simulink model "model"  (R2016a)
(part 4 of 5)

  bus264 : powerlib/Measurements/Load Flow Bus  LConnTagsString=a  Phases=single  Connectors=on one side  ID=bus264  Vbase=400000  Vref=1  Vangle=0  VLF=1  VLFb=1  VLFc=1  angleLF=0  angleLFb=0  angleLFc=0
      settings: AttributesFormatString=|
      | %<ID>
      | %<Vbase>V
      | %<VLF>pu
      | %<angleLF>deg.
      | %<Name>
  bus265 : powerlib/Measurements/Load Flow Bus  LConnTagsString=a  Phases=single  Connectors=on one side  ID=bus265  Vbase=400000  Vref=1  Vangle=0  VLF=1  VLFb=1  VLFc=1  angleLF=0  angleLFb=0  angleLFc=0
      settings: AttributesFormatString=|
      | %<ID>
      | %<Vbase>V
      | %<VLF>pu
      | %<angleLF>deg.
      | %<Name>
  bus266 : powerlib/Measurements/Load Flow Bus  LConnTagsString=a  Phases=single  Connectors=on one side  ID=bus266  Vbase=400000  Vref=1  Vangle=0  VLF=1  VLFb=1  VLFc=1  angleLF=0  angleLFb=0  angleLFc=0
      settings: AttributesFormatString=|
      | %<ID>
      | %<Vbase>V
      | %<VLF>pu
      | %<angleLF>deg.
      | %<Name>
  bus267 : powerlib/Measurements/Load Flow Bus  LConnTagsString=a  Phases=single  Connectors=on one side  ID=bus267  Vbase=400000  Vref=1  Vangle=0  VLF=1  VLFb=1  VLFc=1  angleLF=0  angleLFb=0  angleLFc=0
      settings: AttributesFormatString=|
      | %<ID>
      | %<Vbase>V
      | %<VLF>pu
      | %<angleLF>deg.
      | %<Name>
  bus268 : powerlib/Measurements/Load Flow Bus  LConnTagsString=a  Phases=single  Connectors=on one side  ID=bus268  Vbase=400000  Vref=1  Vangle=0  VLF=1  VLFb=1  VLFc=1  angleLF=0  angleLFb=0  angleLFc=0
      settings: AttributesFormatString=|
      | %<ID>
      | %<Vbase>V
      | %<VLF>pu
      | %<angleLF>deg.
      | %<Name>
  bus269 : powerlib/Measurements/Load Flow Bus  LConnTagsString=a  Phases=single  Connectors=on one side  ID=bus269  Vbase=400000  Vref=1  Vangle=0  VLF=1  VLFb=1  VLFc=1  angleLF=0  angleLFb=0  angleLFc=0
      settings: AttributesFormatString=|
      | %<ID>
      | %<Vbase>V
      | %<VLF>pu
      | %<angleLF>deg.
      | %<Name>
  bus27 : powerlib/Measurements/Load Flow Bus  LConnTagsString=a  Phases=single  Connectors=on one side  ID=bus27  Vbase=400000  Vref=1  Vangle=0  VLF=1  VLFb=1  VLFc=1  angleLF=0  angleLFb=0  angleLFc=0
      settings: AttributesFormatString=|
      | %<ID>
      | %<Vbase>V
      | %<VLF>pu
      | %<angleLF>deg.
      | %<Name>
  bus270 : powerlib/Measurements/Load Flow Bus  LConnTagsString=a  Phases=single  Connectors=on one side  ID=bus270  Vbase=400000  Vref=1  Vangle=0  VLF=1  VLFb=1  VLFc=1  angleLF=0  angleLFb=0  angleLFc=0
      settings: AttributesFormatString=|
      | %<ID>
      | %<Vbase>V
      | %<VLF>pu
      | %<angleLF>deg.
      | %<Name>
  bus271 : powerlib/Measurements/Load Flow Bus  LConnTagsString=a  Phases=single  Connectors=on one side  ID=bus271  Vbase=400000  Vref=1  Vangle=0  VLF=1  VLFb=1  VLFc=1  angleLF=0  angleLFb=0  angleLFc=0
      settings: AttributesFormatString=|
      | %<ID>
      | %<Vbase>V
      | %<VLF>pu
      | %<angleLF>deg.
      | %<Name>
  bus272 : powerlib/Measurements/Load Flow Bus  LConnTagsString=a  Phases=single  Connectors=on one side  ID=bus272  Vbase=400000  Vref=1  Vangle=0  VLF=1  VLFb=1  VLFc=1  angleLF=0  angleLFb=0  angleLFc=0
      settings: AttributesFormatString=|
      | %<ID>
      | %<Vbase>V
      | %<VLF>pu
      | %<angleLF>deg.
      | %<Name>
  bus273 : powerlib/Measurements/Load Flow Bus  LConnTagsString=a  Phases=single  Connectors=on one side  ID=bus273  Vbase=400000  Vref=1  Vangle=0  VLF=1  VLFb=1  VLFc=1  angleLF=0  angleLFb=0  angleLFc=0
      settings: AttributesFormatString=|
      | %<ID>
      | %<Vbase>V
      | %<VLF>pu
      | %<angleLF>deg.
      | %<Name>
  bus274 : powerlib/Measurements/Load Flow Bus  LConnTagsString=a  Phases=single  Connectors=on one side  ID=bus274  Vbase=400000  Vref=1  Vangle=0  VLF=1  VLFb=1  VLFc=1  angleLF=0  angleLFb=0  angleLFc=0
      settings: AttributesFormatString=|
      | %<ID>
      | %<Vbase>V
      | %<VLF>pu
      | %<angleLF>deg.
      | %<Name>
  bus275 : powerlib/Measurements/Load Flow Bus  LConnTagsString=a  Phases=single  Connectors=on one side  ID=bus275  Vbase=400000  Vref=1  Vangle=0  VLF=1  VLFb=1  VLFc=1  angleLF=0  angleLFb=0  angleLFc=0
      settings: AttributesFormatString=|
      | %<ID>
      | %<Vbase>V
      | %<VLF>pu
      | %<angleLF>deg.
      | %<Name>
  bus276 : powerlib/Measurements/Load Flow Bus  LConnTagsString=a  Phases=single  Connectors=on one side  ID=bus276  Vbase=400000  Vref=1  Vangle=0  VLF=1  VLFb=1  VLFc=1  angleLF=0  angleLFb=0  angleLFc=0
      settings: AttributesFormatString=|
      | %<ID>
      | %<Vbase>V
      | %<VLF>pu
      | %<angleLF>deg.
      | %<Name>
  bus277 : powerlib/Measurements/Load Flow Bus  LConnTagsString=a  Phases=single  Connectors=on one side  ID=bus277  Vbase=400000  Vref=1  Vangle=0  VLF=1  VLFb=1  VLFc=1  angleLF=0  angleLFb=0  angleLFc=0
      settings: AttributesFormatString=|
      | %<ID>
      | %<Vbase>V
      | %<VLF>pu
      | %<angleLF>deg.
      | %<Name>
  bus278 : powerlib/Measurements/Load Flow Bus  LConnTagsString=a  Phases=single  Connectors=on one side  ID=bus278  Vbase=400000  Vref=1  Vangle=0  VLF=1  VLFb=1  VLFc=1  angleLF=0  angleLFb=0  angleLFc=0
      settings: AttributesFormatString=|
      | %<ID>
      | %<Vbase>V
      | %<VLF>pu
      | %<angleLF>deg.
      | %<Name>
  bus279 : powerlib/Measurements/Load Flow Bus  LConnTagsString=a  Phases=single  Connectors=on one side  ID=bus279  Vbase=400000  Vref=1  Vangle=0  VLF=1  VLFb=1  VLFc=1  angleLF=0  angleLFb=0  angleLFc=0
      settings: AttributesFormatString=|
      | %<ID>
      | %<Vbase>V
      | %<VLF>pu
      | %<angleLF>deg.
      | %<Name>
  bus28 : powerlib/Measurements/Load Flow Bus  LConnTagsString=a  Phases=single  Connectors=on one side  ID=bus28  Vbase=400000  Vref=1  Vangle=0  VLF=1  VLFb=1  VLFc=1  angleLF=0  angleLFb=0  angleLFc=0
      settings: AttributesFormatString=|
      | %<ID>
      | %<Vbase>V
      | %<VLF>pu
      | %<angleLF>deg.
      | %<Name>
  bus280 : powerlib/Measurements/Load Flow Bus  LConnTagsString=a  Phases=single  Connectors=on one side  ID=bus280  Vbase=400000  Vref=1  Vangle=0  VLF=1  VLFb=1  VLFc=1  angleLF=0  angleLFb=0  angleLFc=0
      settings: AttributesFormatString=|
      | %<ID>
      | %<Vbase>V
      | %<VLF>pu
      | %<angleLF>deg.
      | %<Name>
  bus281 : powerlib/Measurements/Load Flow Bus  LConnTagsString=a  Phases=single  Connectors=on one side  ID=bus281  Vbase=400000  Vref=1  Vangle=0  VLF=1  VLFb=1  VLFc=1  angleLF=0  angleLFb=0  angleLFc=0
      settings: AttributesFormatString=|
      | %<ID>
      | %<Vbase>V
      | %<VLF>pu
      | %<angleLF>deg.
      | %<Name>
  bus282 : powerlib/Measurements/Load Flow Bus  LConnTagsString=a  Phases=single  Connectors=on one side  ID=bus282  Vbase=400000  Vref=1  Vangle=0  VLF=1  VLFb=1  VLFc=1  angleLF=0  angleLFb=0  angleLFc=0
      settings: AttributesFormatString=|
      | %<ID>
      | %<Vbase>V
      | %<VLF>pu
      | %<angleLF>deg.
      | %<Name>
  bus283 : powerlib/Measurements/Load Flow Bus  LConnTagsString=a  Phases=single  Connectors=on one side  ID=bus283  Vbase=400000  Vref=1  Vangle=0  VLF=1  VLFb=1  VLFc=1  angleLF=0  angleLFb=0  angleLFc=0
      settings: AttributesFormatString=|
      | %<ID>
      | %<Vbase>V
      | %<VLF>pu
      | %<angleLF>deg.
      | %<Name>
  bus284 : powerlib/Measurements/Load Flow Bus  LConnTagsString=a  Phases=single  Connectors=on one side  ID=bus284  Vbase=400000  Vref=1  Vangle=0  VLF=1  VLFb=1  VLFc=1  angleLF=0  angleLFb=0  angleLFc=0
      settings: AttributesFormatString=|
      | %<ID>
      | %<Vbase>V
      | %<VLF>pu
      | %<angleLF>deg.
      | %<Name>
  bus285 : powerlib/Measurements/Load Flow Bus  LConnTagsString=a  Phases=single  Connectors=on one side  ID=bus285  Vbase=400000  Vref=1  Vangle=0  VLF=1  VLFb=1  VLFc=1  angleLF=0  angleLFb=0  angleLFc=0
      settings: AttributesFormatString=|
      | %<ID>
      | %<Vbase>V
      | %<VLF>pu
      | %<angleLF>deg.
      | %<Name>
  bus286 : powerlib/Measurements/Load Flow Bus  LConnTagsString=a  Phases=single  Connectors=on one side  ID=bus286  Vbase=400000  Vref=1  Vangle=0  VLF=1  VLFb=1  VLFc=1  angleLF=0  angleLFb=0  angleLFc=0
      settings: AttributesFormatString=|
      | %<ID>
      | %<Vbase>V
      | %<VLF>pu
      | %<angleLF>deg.
      | %<Name>
  bus287 : powerlib/Measurements/Load Flow Bus  LConnTagsString=a  Phases=single  Connectors=on one side  ID=bus287  Vbase=400000  Vref=1  Vangle=0  VLF=1  VLFb=1  VLFc=1  angleLF=0  angleLFb=0  angleLFc=0
      settings: AttributesFormatString=|
      | %<ID>
      | %<Vbase>V
      | %<VLF>pu
      | %<angleLF>deg.
      | %<Name>
  bus288 : powerlib/Measurements/Load Flow Bus  LConnTagsString=a  Phases=single  Connectors=on one side  ID=bus288  Vbase=400000  Vref=1  Vangle=0  VLF=1  VLFb=1  VLFc=1  angleLF=0  angleLFb=0  angleLFc=0
      settings: AttributesFormatString=|
      | %<ID>
      | %<Vbase>V
      | %<VLF>pu
      | %<angleLF>deg.
      | %<Name>
  bus289 : powerlib/Measurements/Load Flow Bus  LConnTagsString=a  Phases=single  Connectors=on one side  ID=bus289  Vbase=400000  Vref=1  Vangle=0  VLF=1  VLFb=1  VLFc=1  angleLF=0  angleLFb=0  angleLFc=0
      settings: AttributesFormatString=|
      | %<ID>
      | %<Vbase>V
      | %<VLF>pu
      | %<angleLF>deg.
      | %<Name>
  bus29 : powerlib/Measurements/Load Flow Bus  LConnTagsString=a  Phases=single  Connectors=on one side  ID=bus29  Vbase=400000  Vref=1  Vangle=0  VLF=1  VLFb=1  VLFc=1  angleLF=0  angleLFb=0  angleLFc=0
      settings: AttributesFormatString=|
      | %<ID>
      | %<Vbase>V
      | %<VLF>pu
      | %<angleLF>deg.
      | %<Name>
  bus290 : powerlib/Measurements/Load Flow Bus  LConnTagsString=a  Phases=single  Connectors=on one side  ID=bus290  Vbase=400000  Vref=1  Vangle=0  VLF=1  VLFb=1  VLFc=1  angleLF=0  angleLFb=0  angleLFc=0
      settings: AttributesFormatString=|
      | %<ID>
      | %<Vbase>V
      | %<VLF>pu
      | %<angleLF>deg.
      | %<Name>
  bus291 : powerlib/Measurements/Load Flow Bus  LConnTagsString=a  Phases=single  Connectors=on one side  ID=bus291  Vbase=400000  Vref=1  Vangle=0  VLF=1  VLFb=1  VLFc=1  angleLF=0  angleLFb=0  angleLFc=0
      settings: AttributesFormatString=|
      | %<ID>
      | %<Vbase>V
      | %<VLF>pu
      | %<angleLF>deg.
      | %<Name>
  bus292 : powerlib/Measurements/Load Flow Bus  LConnTagsString=a  Phases=single  Connectors=on one side  ID=bus292  Vbase=400000  Vref=1  Vangle=0  VLF=1  VLFb=1  VLFc=1  angleLF=0  angleLFb=0  angleLFc=0
      settings: AttributesFormatString=|
      | %<ID>
      | %<Vbase>V
      | %<VLF>pu
      | %<angleLF>deg.
      | %<Name>
  bus293 : powerlib/Measurements/Load Flow Bus  LConnTagsString=a  Phases=single  Connectors=on one side  ID=bus293  Vbase=400000  Vref=1  Vangle=0  VLF=1  VLFb=1  VLFc=1  angleLF=0  angleLFb=0  angleLFc=0
      settings: AttributesFormatString=|
      | %<ID>
      | %<Vbase>V
      | %<VLF>pu
      | %<angleLF>deg.
      | %<Name>
  bus294 : powerlib/Measurements/Load Flow Bus  LConnTagsString=a  Phases=single  Connectors=on one side  ID=bus294  Vbase=400000  Vref=1  Vangle=0  VLF=1  VLFb=1  VLFc=1  angleLF=0  angleLFb=0  angleLFc=0
      settings: AttributesFormatString=|
      | %<ID>
      | %<Vbase>V
      | %<VLF>pu
      | %<angleLF>deg.
      | %<Name>
  bus295 : powerlib/Measurements/Load Flow Bus  LConnTagsString=a  Phases=single  Connectors=on one side  ID=bus295  Vbase=400000  Vref=1  Vangle=0  VLF=1  VLFb=1  VLFc=1  angleLF=0  angleLFb=0  angleLFc=0
      settings: AttributesFormatString=|
      | %<ID>
      | %<Vbase>V
      | %<VLF>pu
      | %<angleLF>deg.
      | %<Name>
  bus296 : powerlib/Measurements/Load Flow Bus  LConnTagsString=a  Phases=single  Connectors=on one side  ID=bus296  Vbase=400000  Vref=1  Vangle=0  VLF=1  VLFb=1  VLFc=1  angleLF=0  angleLFb=0  angleLFc=0
      settings: AttributesFormatString=|
      | %<ID>
      | %<Vbase>V
      | %<VLF>pu
      | %<angleLF>deg.
      | %<Name>
  bus297 : powerlib/Measurements/Load Flow Bus  LConnTagsString=a  Phases=single  Connectors=on one side  ID=bus297  Vbase=400000  Vref=1  Vangle=0  VLF=1  VLFb=1  VLFc=1  angleLF=0  angleLFb=0  angleLFc=0
      settings: AttributesFormatString=|
      | %<ID>
      | %<Vbase>V
      | %<VLF>pu
      | %<angleLF>deg.
      | %<Name>
  bus298 : powerlib/Measurements/Load Flow Bus  LConnTagsString=a  Phases=single  Connectors=on one side  ID=bus298  Vbase=400000  Vref=1  Vangle=0  VLF=1  VLFb=1  VLFc=1  angleLF=0  angleLFb=0  angleLFc=0
      settings: AttributesFormatString=|
      | %<ID>
      | %<Vbase>V
      | %<VLF>pu
      | %<angleLF>deg.
      | %<Name>
  bus299 : powerlib/Measurements/Load Flow Bus  LConnTagsString=a  Phases=single  Connectors=on one side  ID=bus299  Vbase=400000  Vref=1  Vangle=0  VLF=1  VLFb=1  VLFc=1  angleLF=0  angleLFb=0  angleLFc=0
      settings: AttributesFormatString=|
      | %<ID>
      | %<Vbase>V
      | %<VLF>pu
      | %<angleLF>deg.
      | %<Name>
  bus3 : powerlib/Measurements/Load Flow Bus  LConnTagsString=a  Phases=single  Connectors=on one side  ID=bus3  Vbase=400000  Vref=1  Vangle=0  VLF=1  VLFb=1  VLFc=1  angleLF=0  angleLFb=0  angleLFc=0
      settings: AttributesFormatString=|
      | %<ID>
      | %<Vbase>V
      | %<VLF>pu
      | %<angleLF>deg.
      | %<Name>
  bus30 : powerlib/Measurements/Load Flow Bus  LConnTagsString=a  Phases=single  Connectors=on one side  ID=bus30  Vbase=400000  Vref=1  Vangle=0  VLF=1  VLFb=1  VLFc=1  angleLF=0  angleLFb=0  angleLFc=0
      settings: AttributesFormatString=|
      | %<ID>
      | %<Vbase>V
      | %<VLF>pu
      | %<angleLF>deg.
      | %<Name>
  bus300 : powerlib/Measurements/Load Flow Bus  LConnTagsString=a  Phases=single  Connectors=on one side  ID=bus300  Vbase=400000  Vref=1  Vangle=0  VLF=1  VLFb=1  VLFc=1  angleLF=0  angleLFb=0  angleLFc=0
      settings: AttributesFormatString=|
      | %<ID>
      | %<Vbase>V
      | %<VLF>pu
      | %<angleLF>deg.
      | %<Name>
  bus301 : powerlib/Measurements/Load Flow Bus  LConnTagsString=a  Phases=single  Connectors=on one side  ID=bus301  Vbase=400000  Vref=1  Vangle=0  VLF=1  VLFb=1  VLFc=1  angleLF=0  angleLFb=0  angleLFc=0
      settings: AttributesFormatString=|
      | %<ID>
      | %<Vbase>V
      | %<VLF>pu
      | %<angleLF>deg.
      | %<Name>
  bus302 : powerlib/Measurements/Load Flow Bus  LConnTagsString=a  Phases=single  Connectors=on one side  ID=bus302  Vbase=400000  Vref=1  Vangle=0  VLF=1  VLFb=1  VLFc=1  angleLF=0  angleLFb=0  angleLFc=0
      settings: AttributesFormatString=|
      | %<ID>
      | %<Vbase>V
      | %<VLF>pu
      | %<angleLF>deg.
      | %<Name>
  bus303 : powerlib/Measurements/Load Flow Bus  LConnTagsString=a  Phases=single  Connectors=on one side  ID=bus303  Vbase=400000  Vref=1  Vangle=0  VLF=1  VLFb=1  VLFc=1  angleLF=0  angleLFb=0  angleLFc=0
      settings: AttributesFormatString=|
      | %<ID>
      | %<Vbase>V
      | %<VLF>pu
      | %<angleLF>deg.
      | %<Name>
  bus304 : powerlib/Measurements/Load Flow Bus  LConnTagsString=a  Phases=single  Connectors=on one side  ID=bus304  Vbase=400000  Vref=1  Vangle=0  VLF=1  VLFb=1  VLFc=1  angleLF=0  angleLFb=0  angleLFc=0
      settings: AttributesFormatString=|
      | %<ID>
      | %<Vbase>V
      | %<VLF>pu
      | %<angleLF>deg.
      | %<Name>
  bus305 : powerlib/Measurements/Load Flow Bus  LConnTagsString=a  Phases=single  Connectors=on one side  ID=bus305  Vbase=400000  Vref=1  Vangle=0  VLF=1  VLFb=1  VLFc=1  angleLF=0  angleLFb=0  angleLFc=0
      settings: AttributesFormatString=|
      | %<ID>
      | %<Vbase>V
      | %<VLF>pu
      | %<angleLF>deg.
      | %<Name>
  bus306 : powerlib/Measurements/Load Flow Bus  LConnTagsString=a  Phases=single  Connectors=on one side  ID=bus306  Vbase=400000  Vref=1  Vangle=0  VLF=1  VLFb=1  VLFc=1  angleLF=0  angleLFb=0  angleLFc=0
      settings: AttributesFormatString=|
      | %<ID>
      | %<Vbase>V
      | %<VLF>pu
      | %<angleLF>deg.
      | %<Name>
  bus307 : powerlib/Measurements/Load Flow Bus  LConnTagsString=a  Phases=single  Connectors=on one side  ID=bus307  Vbase=400000  Vref=1  Vangle=0  VLF=1  VLFb=1  VLFc=1  angleLF=0  angleLFb=0  angleLFc=0
      settings: AttributesFormatString=|
      | %<ID>
      | %<Vbase>V
      | %<VLF>pu
      | %<angleLF>deg.
      | %<Name>
  bus308 : powerlib/Measurements/Load Flow Bus  LConnTagsString=a  Phases=single  Connectors=on one side  ID=bus308  Vbase=400000  Vref=1  Vangle=0  VLF=1  VLFb=1  VLFc=1  angleLF=0  angleLFb=0  angleLFc=0
      settings: AttributesFormatString=|
      | %<ID>
      | %<Vbase>V
      | %<VLF>pu
      | %<angleLF>deg.
      | %<Name>
  bus309 : powerlib/Measurements/Load Flow Bus  LConnTagsString=a  Phases=single  Connectors=on one side  ID=bus309  Vbase=400000  Vref=1  Vangle=0  VLF=1  VLFb=1  VLFc=1  angleLF=0  angleLFb=0  angleLFc=0
      settings: AttributesFormatString=|
      | %<ID>
      | %<Vbase>V
      | %<VLF>pu
      | %<angleLF>deg.
      | %<Name>
  bus31 : powerlib/Measurements/Load Flow Bus  LConnTagsString=a  Phases=single  Connectors=on one side  ID=bus31  Vbase=400000  Vref=1  Vangle=0  VLF=1  VLFb=1  VLFc=1  angleLF=0  angleLFb=0  angleLFc=0
      settings: AttributesFormatString=|
      | %<ID>
      | %<Vbase>V
      | %<VLF>pu
      | %<angleLF>deg.
      | %<Name>
  bus310 : powerlib/Measurements/Load Flow Bus  LConnTagsString=a  Phases=single  Connectors=on one side  ID=bus310  Vbase=400000  Vref=1  Vangle=0  VLF=1  VLFb=1  VLFc=1  angleLF=0  angleLFb=0  angleLFc=0
      settings: AttributesFormatString=|
      | %<ID>
      | %<Vbase>V
      | %<VLF>pu
      | %<angleLF>deg.
      | %<Name>
  bus311 : powerlib/Measurements/Load Flow Bus  LConnTagsString=a  Phases=single  Connectors=on one side  ID=bus311  Vbase=400000  Vref=1  Vangle=0  VLF=1  VLFb=1  VLFc=1  angleLF=0  angleLFb=0  angleLFc=0
      settings: AttributesFormatString=|
      | %<ID>
      | %<Vbase>V
      | %<VLF>pu
      | %<angleLF>deg.
      | %<Name>
  bus312 : powerlib/Measurements/Load Flow Bus  LConnTagsString=a  Phases=single  Connectors=on one side  ID=bus312  Vbase=400000  Vref=1  Vangle=0  VLF=1  VLFb=1  VLFc=1  angleLF=0  angleLFb=0  angleLFc=0
      settings: AttributesFormatString=|
      | %<ID>
      | %<Vbase>V
      | %<VLF>pu
      | %<angleLF>deg.
      | %<Name>
  bus313 : powerlib/Measurements/Load Flow Bus  LConnTagsString=a  Phases=single  Connectors=on one side  ID=bus313  Vbase=400000  Vref=1  Vangle=0  VLF=1  VLFb=1  VLFc=1  angleLF=0  angleLFb=0  angleLFc=0
      settings: AttributesFormatString=|
      | %<ID>
      | %<Vbase>V
      | %<VLF>pu
      | %<angleLF>deg.
      | %<Name>
  bus314 : powerlib/Measurements/Load Flow Bus  LConnTagsString=a  Phases=single  Connectors=on one side  ID=bus314  Vbase=400000  Vref=1  Vangle=0  VLF=1  VLFb=1  VLFc=1  angleLF=0  angleLFb=0  angleLFc=0
      settings: AttributesFormatString=|
      | %<ID>
      | %<Vbase>V
      | %<VLF>pu
      | %<angleLF>deg.
      | %<Name>
  bus315 : powerlib/Measurements/Load Flow Bus  LConnTagsString=a  Phases=single  Connectors=on one side  ID=bus315  Vbase=400000  Vref=1  Vangle=0  VLF=1  VLFb=1  VLFc=1  angleLF=0  angleLFb=0  angleLFc=0
      settings: AttributesFormatString=|
      | %<ID>
      | %<Vbase>V
      | %<VLF>pu
      | %<angleLF>deg.
      | %<Name>
  bus316 : powerlib/Measurements/Load Flow Bus  LConnTagsString=a  Phases=single  Connectors=on one side  ID=bus316  Vbase=400000  Vref=1  Vangle=0  VLF=1  VLFb=1  VLFc=1  angleLF=0  angleLFb=0  angleLFc=0
      settings: AttributesFormatString=|
      | %<ID>
      | %<Vbase>V
      | %<VLF>pu
      | %<angleLF>deg.
      | %<Name>
  bus317 : powerlib/Measurements/Load Flow Bus  LConnTagsString=a  Phases=single  Connectors=on one side  ID=bus317  Vbase=400000  Vref=1  Vangle=0  VLF=1  VLFb=1  VLFc=1  angleLF=0  angleLFb=0  angleLFc=0
      settings: AttributesFormatString=|
      | %<ID>
      | %<Vbase>V
      | %<VLF>pu
      | %<angleLF>deg.
      | %<Name>
  bus318 : powerlib/Measurements/Load Flow Bus  LConnTagsString=a  Phases=single  Connectors=on one side  ID=bus318  Vbase=400000  Vref=1  Vangle=0  VLF=1  VLFb=1  VLFc=1  angleLF=0  angleLFb=0  angleLFc=0
      settings: AttributesFormatString=|
      | %<ID>
      | %<Vbase>V
      | %<VLF>pu
      | %<angleLF>deg.
      | %<Name>
  bus319 : powerlib/Measurements/Load Flow Bus  LConnTagsString=a  Phases=single  Connectors=on one side  ID=bus319  Vbase=400000  Vref=1  Vangle=0  VLF=1  VLFb=1  VLFc=1  angleLF=0  angleLFb=0  angleLFc=0
      settings: AttributesFormatString=|
      | %<ID>
      | %<Vbase>V
      | %<VLF>pu
      | %<angleLF>deg.
      | %<Name>
  bus32 : powerlib/Measurements/Load Flow Bus  LConnTagsString=a  Phases=single  Connectors=on one side  ID=bus32  Vbase=400000  Vref=1  Vangle=0  VLF=1  VLFb=1  VLFc=1  angleLF=0  angleLFb=0  angleLFc=0
      settings: AttributesFormatString=|
      | %<ID>
      | %<Vbase>V
      | %<VLF>pu
      | %<angleLF>deg.
      | %<Name>
  bus320 : powerlib/Measurements/Load Flow Bus  LConnTagsString=a  Phases=single  Connectors=on one side  ID=bus320  Vbase=400000  Vref=1  Vangle=0  VLF=1  VLFb=1  VLFc=1  angleLF=0  angleLFb=0  angleLFc=0
      settings: AttributesFormatString=|
      | %<ID>
      | %<Vbase>V
      | %<VLF>pu
      | %<angleLF>deg.
      | %<Name>
  bus321 : powerlib/Measurements/Load Flow Bus  LConnTagsString=a  Phases=single  Connectors=on one side  ID=bus321  Vbase=400000  Vref=1  Vangle=0  VLF=1  VLFb=1  VLFc=1  angleLF=0  angleLFb=0  angleLFc=0
      settings: AttributesFormatString=|
      | %<ID>
      | %<Vbase>V
      | %<VLF>pu
      | %<angleLF>deg.
      | %<Name>
  bus322 : powerlib/Measurements/Load Flow Bus  LConnTagsString=a  Phases=single  Connectors=on one side  ID=bus322  Vbase=400000  Vref=1  Vangle=0  VLF=1  VLFb=1  VLFc=1  angleLF=0  angleLFb=0  angleLFc=0
      settings: AttributesFormatString=|
      | %<ID>
      | %<Vbase>V
      | %<VLF>pu
      | %<angleLF>deg.
      | %<Name>
  bus323 : powerlib/Measurements/Load Flow Bus  LConnTagsString=a  Phases=single  Connectors=on one side  ID=bus323  Vbase=400000  Vref=1  Vangle=0  VLF=1  VLFb=1  VLFc=1  angleLF=0  angleLFb=0  angleLFc=0
      settings: AttributesFormatString=|
      | %<ID>
      | %<Vbase>V
      | %<VLF>pu
      | %<angleLF>deg.
      | %<Name>
  bus324 : powerlib/Measurements/Load Flow Bus  LConnTagsString=a  Phases=single  Connectors=on one side  ID=bus324  Vbase=400000  Vref=1  Vangle=0  VLF=1  VLFb=1  VLFc=1  angleLF=0  angleLFb=0  angleLFc=0
      settings: AttributesFormatString=|
      | %<ID>
      | %<Vbase>V
      | %<VLF>pu
      | %<angleLF>deg.
      | %<Name>
  bus325 : powerlib/Measurements/Load Flow Bus  LConnTagsString=a  Phases=single  Connectors=on one side  ID=bus325  Vbase=400000  Vref=1  Vangle=0  VLF=1  VLFb=1  VLFc=1  angleLF=0  angleLFb=0  angleLFc=0
      settings: AttributesFormatString=|
      | %<ID>
      | %<Vbase>V
      | %<VLF>pu
      | %<angleLF>deg.
      | %<Name>
  bus326 : powerlib/Measurements/Load Flow Bus  LConnTagsString=a  Phases=single  Connectors=on one side  ID=bus326  Vbase=400000  Vref=1  Vangle=0  VLF=1  VLFb=1  VLFc=1  angleLF=0  angleLFb=0  angleLFc=0
      settings: AttributesFormatString=|
      | %<ID>
      | %<Vbase>V
      | %<VLF>pu
      | %<angleLF>deg.
      | %<Name>
  bus327 : powerlib/Measurements/Load Flow Bus  LConnTagsString=a  Phases=single  Connectors=on one side  ID=bus327  Vbase=400000  Vref=1  Vangle=0  VLF=1  VLFb=1  VLFc=1  angleLF=0  angleLFb=0  angleLFc=0
      settings: AttributesFormatString=|
      | %<ID>
      | %<Vbase>V
      | %<VLF>pu
      | %<angleLF>deg.
      | %<Name>
  bus328 : powerlib/Measurements/Load Flow Bus  LConnTagsString=a  Phases=single  Connectors=on one side  ID=bus328  Vbase=400000  Vref=1  Vangle=0  VLF=1  VLFb=1  VLFc=1  angleLF=0  angleLFb=0  angleLFc=0
      settings: AttributesFormatString=|
      | %<ID>
      | %<Vbase>V
      | %<VLF>pu
      | %<angleLF>deg.
      | %<Name>
  bus329 : powerlib/Measurements/Load Flow Bus  LConnTagsString=a  Phases=single  Connectors=on one side  ID=bus329  Vbase=400000  Vref=1  Vangle=0  VLF=1  VLFb=1  VLFc=1  angleLF=0  angleLFb=0  angleLFc=0
      settings: AttributesFormatString=|
      | %<ID>
      | %<Vbase>V
      | %<VLF>pu
      | %<angleLF>deg.
      | %<Name>
  bus33 : powerlib/Measurements/Load Flow Bus  LConnTagsString=a  Phases=single  Connectors=on one side  ID=bus33  Vbase=400000  Vref=1  Vangle=0  VLF=1  VLFb=1  VLFc=1  angleLF=0  angleLFb=0  angleLFc=0
      settings: AttributesFormatString=|
      | %<ID>
      | %<Vbase>V
      | %<VLF>pu
      | %<angleLF>deg.
      | %<Name>
  bus330 : powerlib/Measurements/Load Flow Bus  LConnTagsString=a  Phases=single  Connectors=on one side  ID=bus330  Vbase=400000  Vref=1  Vangle=0  VLF=1  VLFb=1  VLFc=1  angleLF=0  angleLFb=0  angleLFc=0
      settings: AttributesFormatString=|
      | %<ID>
      | %<Vbase>V
      | %<VLF>pu
      | %<angleLF>deg.
      | %<Name>
  bus331 : powerlib/Measurements/Load Flow Bus  LConnTagsString=a  Phases=single  Connectors=on one side  ID=bus331  Vbase=400000  Vref=1  Vangle=0  VLF=1  VLFb=1  VLFc=1  angleLF=0  angleLFb=0  angleLFc=0
      settings: AttributesFormatString=|
      | %<ID>
      | %<Vbase>V
      | %<VLF>pu
      | %<angleLF>deg.
      | %<Name>
  bus332 : powerlib/Measurements/Load Flow Bus  LConnTagsString=a  Phases=single  Connectors=on one side  ID=bus332  Vbase=400000  Vref=1  Vangle=0  VLF=1  VLFb=1  VLFc=1  angleLF=0  angleLFb=0  angleLFc=0
      settings: AttributesFormatString=|
      | %<ID>
      | %<Vbase>V
      | %<VLF>pu
      | %<angleLF>deg.
      | %<Name>
  bus333 : powerlib/Measurements/Load Flow Bus  LConnTagsString=a  Phases=single  Connectors=on one side  ID=bus333  Vbase=400000  Vref=1  Vangle=0  VLF=1  VLFb=1  VLFc=1  angleLF=0  angleLFb=0  angleLFc=0
      settings: AttributesFormatString=|
      | %<ID>
      | %<Vbase>V
      | %<VLF>pu
      | %<angleLF>deg.
      | %<Name>
  bus334 : powerlib/Measurements/Load Flow Bus  LConnTagsString=a  Phases=single  Connectors=on one side  ID=bus334  Vbase=400000  Vref=1  Vangle=0  VLF=1  VLFb=1  VLFc=1  angleLF=0  angleLFb=0  angleLFc=0
      settings: AttributesFormatString=|
      | %<ID>
      | %<Vbase>V
      | %<VLF>pu
      | %<angleLF>deg.
      | %<Name>
  bus335 : powerlib/Measurements/Load Flow Bus  LConnTagsString=a  Phases=single  Connectors=on one side  ID=bus335  Vbase=400000  Vref=1  Vangle=0  VLF=1  VLFb=1  VLFc=1  angleLF=0  angleLFb=0  angleLFc=0
      settings: AttributesFormatString=|
      | %<ID>
      | %<Vbase>V
      | %<VLF>pu
      | %<angleLF>deg.
      | %<Name>
  bus336 : powerlib/Measurements/Load Flow Bus  LConnTagsString=a  Phases=single  Connectors=on one side  ID=bus336  Vbase=400000  Vref=1  Vangle=0  VLF=1  VLFb=1  VLFc=1  angleLF=0  angleLFb=0  angleLFc=0
      settings: AttributesFormatString=|
      | %<ID>
      | %<Vbase>V
      | %<VLF>pu
      | %<angleLF>deg.
      | %<Name>
  bus337 : powerlib/Measurements/Load Flow Bus  LConnTagsString=a  Phases=single  Connectors=on one side  ID=bus337  Vbase=400000  Vref=1  Vangle=0  VLF=1  VLFb=1  VLFc=1  angleLF=0  angleLFb=0  angleLFc=0
      settings: AttributesFormatString=|
      | %<ID>
      | %<Vbase>V
      | %<VLF>pu
      | %<angleLF>deg.
      | %<Name>
  bus338 : powerlib/Measurements/Load Flow Bus  LConnTagsString=a  Phases=single  Connectors=on one side  ID=bus338  Vbase=400000  Vref=1  Vangle=0  VLF=1  VLFb=1  VLFc=1  angleLF=0  angleLFb=0  angleLFc=0
      settings: AttributesFormatString=|
      | %<ID>
      | %<Vbase>V
      | %<VLF>pu
      | %<angleLF>deg.
      | %<Name>
  bus339 : powerlib/Measurements/Load Flow Bus  LConnTagsString=a  Phases=single  Connectors=on one side  ID=bus339  Vbase=400000  Vref=1  Vangle=0  VLF=1  VLFb=1  VLFc=1  angleLF=0  angleLFb=0  angleLFc=0
      settings: AttributesFormatString=|
      | %<ID>
      | %<Vbase>V
      | %<VLF>pu
      | %<angleLF>deg.
      | %<Name>
  bus34 : powerlib/Measurements/Load Flow Bus  LConnTagsString=a  Phases=single  Connectors=on one side  ID=bus34  Vbase=400000  Vref=1  Vangle=0  VLF=1  VLFb=1  VLFc=1  angleLF=0  angleLFb=0  angleLFc=0
      settings: AttributesFormatString=|
      | %<ID>
      | %<Vbase>V
      | %<VLF>pu
      | %<angleLF>deg.
      | %<Name>
  bus340 : powerlib/Measurements/Load Flow Bus  LConnTagsString=a  Phases=single  Connectors=on one side  ID=bus340  Vbase=400000  Vref=1  Vangle=0  VLF=1  VLFb=1  VLFc=1  angleLF=0  angleLFb=0  angleLFc=0
      settings: AttributesFormatString=|
      | %<ID>
      | %<Vbase>V
      | %<VLF>pu
      | %<angleLF>deg.
      | %<Name>
  bus341 : powerlib/Measurements/Load Flow Bus  LConnTagsString=a  Phases=single  Connectors=on one side  ID=bus341  Vbase=400000  Vref=1  Vangle=0  VLF=1  VLFb=1  VLFc=1  angleLF=0  angleLFb=0  angleLFc=0
      settings: AttributesFormatString=|
      | %<ID>
      | %<Vbase>V
      | %<VLF>pu
      | %<angleLF>deg.
      | %<Name>
  bus342 : powerlib/Measurements/Load Flow Bus  LConnTagsString=a  Phases=single  Connectors=on one side  ID=bus342  Vbase=400000  Vref=1  Vangle=0  VLF=1  VLFb=1  VLFc=1  angleLF=0  angleLFb=0  angleLFc=0
      settings: AttributesFormatString=|
      | %<ID>
      | %<Vbase>V
      | %<VLF>pu
      | %<angleLF>deg.
      | %<Name>
  bus343 : powerlib/Measurements/Load Flow Bus  LConnTagsString=a  Phases=single  Connectors=on one side  ID=bus343  Vbase=400000  Vref=1  Vangle=0  VLF=1  VLFb=1  VLFc=1  angleLF=0  angleLFb=0  angleLFc=0
      settings: AttributesFormatString=|
      | %<ID>
      | %<Vbase>V
      | %<VLF>pu
      | %<angleLF>deg.
      | %<Name>
  bus344 : powerlib/Measurements/Load Flow Bus  LConnTagsString=a  Phases=single  Connectors=on one side  ID=bus344  Vbase=400000  Vref=1  Vangle=0  VLF=1  VLFb=1  VLFc=1  angleLF=0  angleLFb=0  angleLFc=0
      settings: AttributesFormatString=|
      | %<ID>
      | %<Vbase>V
      | %<VLF>pu
      | %<angleLF>deg.
      | %<Name>
  bus345 : powerlib/Measurements/Load Flow Bus  LConnTagsString=a  Phases=single  Connectors=on one side  ID=bus345  Vbase=400000  Vref=1  Vangle=0  VLF=1  VLFb=1  VLFc=1  angleLF=0  angleLFb=0  angleLFc=0
      settings: AttributesFormatString=|
      | %<ID>
      | %<Vbase>V
      | %<VLF>pu
      | %<angleLF>deg.
      | %<Name>
  bus346 : powerlib/Measurements/Load Flow Bus  LConnTagsString=a  Phases=single  Connectors=on one side  ID=bus346  Vbase=400000  Vref=1  Vangle=0  VLF=1  VLFb=1  VLFc=1  angleLF=0  angleLFb=0  angleLFc=0
      settings: AttributesFormatString=|
      | %<ID>
      | %<Vbase>V
      | %<VLF>pu
      | %<angleLF>deg.
      | %<Name>
  bus347 : powerlib/Measurements/Load Flow Bus  LConnTagsString=a  Phases=single  Connectors=on one side  ID=bus347  Vbase=400000  Vref=1  Vangle=0  VLF=1  VLFb=1  VLFc=1  angleLF=0  angleLFb=0  angleLFc=0
      settings: AttributesFormatString=|
      | %<ID>
      | %<Vbase>V
      | %<VLF>pu
      | %<angleLF>deg.
      | %<Name>
  bus348 : powerlib/Measurements/Load Flow Bus  LConnTagsString=a  Phases=single  Connectors=on one side  ID=bus348  Vbase=400000  Vref=1  Vangle=0  VLF=1  VLFb=1  VLFc=1  angleLF=0  angleLFb=0  angleLFc=0
      settings: AttributesFormatString=|
      | %<ID>
      | %<Vbase>V
      | %<VLF>pu
      | %<angleLF>deg.
      | %<Name>
  bus349 : powerlib/Measurements/Load Flow Bus  LConnTagsString=a  Phases=single  Connectors=on one side  ID=bus349  Vbase=400000  Vref=1  Vangle=0  VLF=1  VLFb=1  VLFc=1  angleLF=0  angleLFb=0  angleLFc=0
      settings: AttributesFormatString=|
      | %<ID>
      | %<Vbase>V
      | %<VLF>pu
      | %<angleLF>deg.
      | %<Name>
  bus35 : powerlib/Measurements/Load Flow Bus  LConnTagsString=a  Phases=single  Connectors=on one side  ID=bus35  Vbase=400000  Vref=1  Vangle=0  VLF=1  VLFb=1  VLFc=1  angleLF=0  angleLFb=0  angleLFc=0
      settings: AttributesFormatString=|
      | %<ID>
      | %<Vbase>V
      | %<VLF>pu
      | %<angleLF>deg.
      | %<Name>
  bus350 : powerlib/Measurements/Load Flow Bus  LConnTagsString=a  Phases=single  Connectors=on one side  ID=bus350  Vbase=400000  Vref=1  Vangle=0  VLF=1  VLFb=1  VLFc=1  angleLF=0  angleLFb=0  angleLFc=0
      settings: AttributesFormatString=|
      | %<ID>
      | %<Vbase>V
      | %<VLF>pu
      | %<angleLF>deg.
      | %<Name>
  bus351 : powerlib/Measurements/Load Flow Bus  LConnTagsString=a  Phases=single  Connectors=on one side  ID=bus351  Vbase=400000  Vref=1  Vangle=0  VLF=1  VLFb=1  VLFc=1  angleLF=0  angleLFb=0  angleLFc=0
      settings: AttributesFormatString=|
      | %<ID>
      | %<Vbase>V
      | %<VLF>pu
      | %<angleLF>deg.
      | %<Name>
  bus352 : powerlib/Measurements/Load Flow Bus  LConnTagsString=a  Phases=single  Connectors=on one side  ID=bus352  Vbase=400000  Vref=1  Vangle=0  VLF=1  VLFb=1  VLFc=1  angleLF=0  angleLFb=0  angleLFc=0
      settings: AttributesFormatString=|
      | %<ID>
      | %<Vbase>V
      | %<VLF>pu
      | %<angleLF>deg.
      | %<Name>
  bus353 : powerlib/Measurements/Load Flow Bus  LConnTagsString=a  Phases=single  Connectors=on one side  ID=bus353  Vbase=400000  Vref=1  Vangle=0  VLF=1  VLFb=1  VLFc=1  angleLF=0  angleLFb=0  angleLFc=0
      settings: AttributesFormatString=|
      | %<ID>
      | %<Vbase>V
      | %<VLF>pu
      | %<angleLF>deg.
      | %<Name>
  bus354 : powerlib/Measurements/Load Flow Bus  LConnTagsString=a  Phases=single  Connectors=on one side  ID=bus354  Vbase=400000  Vref=1  Vangle=0  VLF=1  VLFb=1  VLFc=1  angleLF=0  angleLFb=0  angleLFc=0
      settings: AttributesFormatString=|
      | %<ID>
      | %<Vbase>V
      | %<VLF>pu
      | %<angleLF>deg.
      | %<Name>
  bus355 : powerlib/Measurements/Load Flow Bus  LConnTagsString=a  Phases=single  Connectors=on one side  ID=bus355  Vbase=400000  Vref=1  Vangle=0  VLF=1  VLFb=1  VLFc=1  angleLF=0  angleLFb=0  angleLFc=0
      settings: AttributesFormatString=|
      | %<ID>
      | %<Vbase>V
      | %<VLF>pu
      | %<angleLF>deg.
      | %<Name>
  bus356 : powerlib/Measurements/Load Flow Bus  LConnTagsString=a  Phases=single  Connectors=on one side  ID=bus356  Vbase=400000  Vref=1  Vangle=0  VLF=1  VLFb=1  VLFc=1  angleLF=0  angleLFb=0  angleLFc=0
      settings: AttributesFormatString=|
      | %<ID>
      | %<Vbase>V
      | %<VLF>pu
      | %<angleLF>deg.
      | %<Name>
  bus357 : powerlib/Measurements/Load Flow Bus  LConnTagsString=a  Phases=single  Connectors=on one side  ID=bus357  Vbase=400000  Vref=1  Vangle=0  VLF=1  VLFb=1  VLFc=1  angleLF=0  angleLFb=0  angleLFc=0
      settings: AttributesFormatString=|
      | %<ID>
      | %<Vbase>V
      | %<VLF>pu
      | %<angleLF>deg.
      | %<Name>
  bus358 : powerlib/Measurements/Load Flow Bus  LConnTagsString=a  Phases=single  Connectors=on one side  ID=bus358  Vbase=400000  Vref=1  Vangle=0  VLF=1  VLFb=1  VLFc=1  angleLF=0  angleLFb=0  angleLFc=0
      settings: AttributesFormatString=|
      | %<ID>
      | %<Vbase>V
      | %<VLF>pu
      | %<angleLF>deg.
      | %<Name>
  bus359 : powerlib/Measurements/Load Flow Bus  LConnTagsString=a  Phases=single  Connectors=on one side  ID=bus359  Vbase=400000  Vref=1  Vangle=0  VLF=1  VLFb=1  VLFc=1  angleLF=0  angleLFb=0  angleLFc=0
      settings: AttributesFormatString=|
      | %<ID>
      | %<Vbase>V
      | %<VLF>pu
      | %<angleLF>deg.
      | %<Name>
  bus36 : powerlib/Measurements/Load Flow Bus  LConnTagsString=a  Phases=single  Connectors=on one side  ID=bus36  Vbase=400000  Vref=1  Vangle=0  VLF=1  VLFb=1  VLFc=1  angleLF=0  angleLFb=0  angleLFc=0
      settings: AttributesFormatString=|
      | %<ID>
      | %<Vbase>V
      | %<VLF>pu
      | %<angleLF>deg.
      | %<Name>
  bus360 : powerlib/Measurements/Load Flow Bus  LConnTagsString=a  Phases=single  Connectors=on one side  ID=bus360  Vbase=400000  Vref=1  Vangle=0  VLF=1  VLFb=1  VLFc=1  angleLF=0  angleLFb=0  angleLFc=0
      settings: AttributesFormatString=|
      | %<ID>
      | %<Vbase>V
      | %<VLF>pu
      | %<angleLF>deg.
      | %<Name>
  bus361 : powerlib/Measurements/Load Flow Bus  LConnTagsString=a  Phases=single  Connectors=on one side  ID=bus361  Vbase=400000  Vref=1  Vangle=0  VLF=1  VLFb=1  VLFc=1  angleLF=0  angleLFb=0  angleLFc=0
      settings: AttributesFormatString=|
      | %<ID>
      | %<Vbase>V
      | %<VLF>pu
      | %<angleLF>deg.
      | %<Name>
  bus362 : powerlib/Measurements/Load Flow Bus  LConnTagsString=a  Phases=single  Connectors=on one side  ID=bus362  Vbase=400000  Vref=1  Vangle=0  VLF=1  VLFb=1  VLFc=1  angleLF=0  angleLFb=0  angleLFc=0
      settings: AttributesFormatString=|
      | %<ID>
      | %<Vbase>V
      | %<VLF>pu
      | %<angleLF>deg.
      | %<Name>
  bus363 : powerlib/Measurements/Load Flow Bus  LConnTagsString=a  Phases=single  Connectors=on one side  ID=bus363  Vbase=400000  Vref=1  Vangle=0  VLF=1  VLFb=1  VLFc=1  angleLF=0  angleLFb=0  angleLFc=0
      settings: AttributesFormatString=|
      | %<ID>
      | %<Vbase>V
      | %<VLF>pu
      | %<angleLF>deg.
      | %<Name>
  bus364 : powerlib/Measurements/Load Flow Bus  LConnTagsString=a  Phases=single  Connectors=on one side  ID=bus364  Vbase=400000  Vref=1  Vangle=0  VLF=1  VLFb=1  VLFc=1  angleLF=0  angleLFb=0  angleLFc=0
      settings: AttributesFormatString=|
      | %<ID>
      | %<Vbase>V
      | %<VLF>pu
      | %<angleLF>deg.
      | %<Name>
  bus365 : powerlib/Measurements/Load Flow Bus  LConnTagsString=a  Phases=single  Connectors=on one side  ID=bus365  Vbase=400000  Vref=1  Vangle=0  VLF=1  VLFb=1  VLFc=1  angleLF=0  angleLFb=0  angleLFc=0
      settings: AttributesFormatString=|
      | %<ID>
      | %<Vbase>V
      | %<VLF>pu
      | %<angleLF>deg.
      | %<Name>
  bus366 : powerlib/Measurements/Load Flow Bus  LConnTagsString=a  Phases=single  Connectors=on one side  ID=bus366  Vbase=400000  Vref=1  Vangle=0  VLF=1  VLFb=1  VLFc=1  angleLF=0  angleLFb=0  angleLFc=0
      settings: AttributesFormatString=|
      | %<ID>
      | %<Vbase>V
      | %<VLF>pu
      | %<angleLF>deg.
      | %<Name>
  bus367 : powerlib/Measurements/Load Flow Bus  LConnTagsString=a  Phases=single  Connectors=on one side  ID=bus367  Vbase=400000  Vref=1  Vangle=0  VLF=1  VLFb=1  VLFc=1  angleLF=0  angleLFb=0  angleLFc=0
      settings: AttributesFormatString=|
      | %<ID>
      | %<Vbase>V
      | %<VLF>pu
      | %<angleLF>deg.
      | %<Name>
  bus368 : powerlib/Measurements/Load Flow Bus  LConnTagsString=a  Phases=single  Connectors=on one side  ID=bus368  Vbase=400000  Vref=1  Vangle=0  VLF=1  VLFb=1  VLFc=1  angleLF=0  angleLFb=0  angleLFc=0
      settings: AttributesFormatString=|
      | %<ID>
      | %<Vbase>V
      | %<VLF>pu
      | %<angleLF>deg.
      | %<Name>
  bus369 : powerlib/Measurements/Load Flow Bus  LConnTagsString=a  Phases=single  Connectors=on one side  ID=bus369  Vbase=400000  Vref=1  Vangle=0  VLF=1  VLFb=1  VLFc=1  angleLF=0  angleLFb=0  angleLFc=0
      settings: AttributesFormatString=|
      | %<ID>
      | %<Vbase>V
      | %<VLF>pu
      | %<angleLF>deg.
      | %<Name>
  bus37 : powerlib/Measurements/Load Flow Bus  LConnTagsString=a  Phases=single  Connectors=on one side  ID=bus37  Vbase=400000  Vref=1  Vangle=0  VLF=1  VLFb=1  VLFc=1  angleLF=0  angleLFb=0  angleLFc=0
      settings: AttributesFormatString=|
      | %<ID>
      | %<Vbase>V
      | %<VLF>pu
      | %<angleLF>deg.
      | %<Name>
  bus370 : powerlib/Measurements/Load Flow Bus  LConnTagsString=a  Phases=single  Connectors=on one side  ID=bus370  Vbase=400000  Vref=1  Vangle=0  VLF=1  VLFb=1  VLFc=1  angleLF=0  angleLFb=0  angleLFc=0
      settings: AttributesFormatString=|
      | %<ID>
      | %<Vbase>V
      | %<VLF>pu
      | %<angleLF>deg.
      | %<Name>
  bus371 : powerlib/Measurements/Load Flow Bus  LConnTagsString=a  Phases=single  Connectors=on one side  ID=bus371  Vbase=400000  Vref=1  Vangle=0  VLF=1  VLFb=1  VLFc=1  angleLF=0  angleLFb=0  angleLFc=0
      settings: AttributesFormatString=|
      | %<ID>
      | %<Vbase>V
      | %<VLF>pu
      | %<angleLF>deg.
      | %<Name>
  bus372 : powerlib/Measurements/Load Flow Bus  LConnTagsString=a  Phases=single  Connectors=on one side  ID=bus372  Vbase=400000  Vref=1  Vangle=0  VLF=1  VLFb=1  VLFc=1  angleLF=0  angleLFb=0  angleLFc=0
      settings: AttributesFormatString=|
      | %<ID>
      | %<Vbase>V
      | %<VLF>pu
      | %<angleLF>deg.
      | %<Name>
  bus373 : powerlib/Measurements/Load Flow Bus  LConnTagsString=a  Phases=single  Connectors=on one side  ID=bus373  Vbase=400000  Vref=1  Vangle=0  VLF=1  VLFb=1  VLFc=1  angleLF=0  angleLFb=0  angleLFc=0
      settings: AttributesFormatString=|
      | %<ID>
      | %<Vbase>V
      | %<VLF>pu
      | %<angleLF>deg.
      | %<Name>
  bus374 : powerlib/Measurements/Load Flow Bus  LConnTagsString=a  Phases=single  Connectors=on one side  ID=bus374  Vbase=400000  Vref=1  Vangle=0  VLF=1  VLFb=1  VLFc=1  angleLF=0  angleLFb=0  angleLFc=0
      settings: AttributesFormatString=|
      | %<ID>
      | %<Vbase>V
      | %<VLF>pu
      | %<angleLF>deg.
      | %<Name>
  bus375 : powerlib/Measurements/Load Flow Bus  LConnTagsString=a  Phases=single  Connectors=on one side  ID=bus375  Vbase=400000  Vref=1  Vangle=0  VLF=1  VLFb=1  VLFc=1  angleLF=0  angleLFb=0  angleLFc=0
      settings: AttributesFormatString=|
      | %<ID>
      | %<Vbase>V
      | %<VLF>pu
      | %<angleLF>deg.
      | %<Name>
  bus376 : powerlib/Measurements/Load Flow Bus  LConnTagsString=a  Phases=single  Connectors=on one side  ID=bus376  Vbase=400000  Vref=1  Vangle=0  VLF=1  VLFb=1  VLFc=1  angleLF=0  angleLFb=0  angleLFc=0
      settings: AttributesFormatString=|
      | %<ID>
      | %<Vbase>V
      | %<VLF>pu
      | %<angleLF>deg.
      | %<Name>
  bus377 : powerlib/Measurements/Load Flow Bus  LConnTagsString=a  Phases=single  Connectors=on one side  ID=bus377  Vbase=400000  Vref=1  Vangle=0  VLF=1  VLFb=1  VLFc=1  angleLF=0  angleLFb=0  angleLFc=0
      settings: AttributesFormatString=|
      | %<ID>
      | %<Vbase>V
      | %<VLF>pu
      | %<angleLF>deg.
      | %<Name>
  bus378 : powerlib/Measurements/Load Flow Bus  LConnTagsString=a  Phases=single  Connectors=on one side  ID=bus378  Vbase=400000  Vref=1  Vangle=0  VLF=1  VLFb=1  VLFc=1  angleLF=0  angleLFb=0  angleLFc=0
      settings: AttributesFormatString=|
      | %<ID>
      | %<Vbase>V
      | %<VLF>pu
      | %<angleLF>deg.
      | %<Name>
  bus379 : powerlib/Measurements/Load Flow Bus  LConnTagsString=a  Phases=single  Connectors=on one side  ID=bus379  Vbase=400000  Vref=1  Vangle=0  VLF=1  VLFb=1  VLFc=1  angleLF=0  angleLFb=0  angleLFc=0
      settings: AttributesFormatString=|
      | %<ID>
      | %<Vbase>V
      | %<VLF>pu
      | %<angleLF>deg.
      | %<Name>
  bus38 : powerlib/Measurements/Load Flow Bus  LConnTagsString=a  Phases=single  Connectors=on one side  ID=bus38  Vbase=400000  Vref=1  Vangle=0  VLF=1  VLFb=1  VLFc=1  angleLF=0  angleLFb=0  angleLFc=0
      settings: AttributesFormatString=|
      | %<ID>
      | %<Vbase>V
      | %<VLF>pu
      | %<angleLF>deg.
      | %<Name>
  bus380 : powerlib/Measurements/Load Flow Bus  LConnTagsString=a  Phases=single  Connectors=on one side  ID=bus380  Vbase=400000  Vref=1  Vangle=0  VLF=1  VLFb=1  VLFc=1  angleLF=0  angleLFb=0  angleLFc=0
      settings: AttributesFormatString=|
      | %<ID>
      | %<Vbase>V
      | %<VLF>pu
      | %<angleLF>deg.
      | %<Name>
  bus381 : powerlib/Measurements/Load Flow Bus  LConnTagsString=a  Phases=single  Connectors=on one side  ID=bus381  Vbase=400000  Vref=1  Vangle=0  VLF=1  VLFb=1  VLFc=1  angleLF=0  angleLFb=0  angleLFc=0
      settings: AttributesFormatString=|
      | %<ID>
      | %<Vbase>V
      | %<VLF>pu
      | %<angleLF>deg.
      | %<Name>
  bus382 : powerlib/Measurements/Load Flow Bus  LConnTagsString=a  Phases=single  Connectors=on one side  ID=bus382  Vbase=400000  Vref=1  Vangle=0  VLF=1  VLFb=1  VLFc=1  angleLF=0  angleLFb=0  angleLFc=0
      settings: AttributesFormatString=|
      | %<ID>
      | %<Vbase>V
      | %<VLF>pu
      | %<angleLF>deg.
      | %<Name>
  bus383 : powerlib/Measurements/Load Flow Bus  LConnTagsString=a  Phases=single  Connectors=on one side  ID=bus383  Vbase=400000  Vref=1  Vangle=0  VLF=1  VLFb=1  VLFc=1  angleLF=0  angleLFb=0  angleLFc=0
      settings: AttributesFormatString=|
      | %<ID>
      | %<Vbase>V
      | %<VLF>pu
      | %<angleLF>deg.
      | %<Name>
  bus384 : powerlib/Measurements/Load Flow Bus  LConnTagsString=a  Phases=single  Connectors=on one side  ID=bus384  Vbase=400000  Vref=1  Vangle=0  VLF=1  VLFb=1  VLFc=1  angleLF=0  angleLFb=0  angleLFc=0
      settings: AttributesFormatString=|
      | %<ID>
      | %<Vbase>V
      | %<VLF>pu
      | %<angleLF>deg.
      | %<Name>
  bus385 : powerlib/Measurements/Load Flow Bus  LConnTagsString=a  Phases=single  Connectors=on one side  ID=bus385  Vbase=400000  Vref=1  Vangle=0  VLF=1  VLFb=1  VLFc=1  angleLF=0  angleLFb=0  angleLFc=0
      settings: AttributesFormatString=|
      | %<ID>
      | %<Vbase>V
      | %<VLF>pu
      | %<angleLF>deg.
      | %<Name>
  bus386 : powerlib/Measurements/Load Flow Bus  LConnTagsString=a  Phases=single  Connectors=on one side  ID=bus386  Vbase=400000  Vref=1  Vangle=0  VLF=1  VLFb=1  VLFc=1  angleLF=0  angleLFb=0  angleLFc=0
      settings: AttributesFormatString=|
      | %<ID>
      | %<Vbase>V
      | %<VLF>pu
      | %<angleLF>deg.
      | %<Name>
  bus387 : powerlib/Measurements/Load Flow Bus  LConnTagsString=a  Phases=single  Connectors=on one side  ID=bus387  Vbase=400000  Vref=1  Vangle=0  VLF=1  VLFb=1  VLFc=1  angleLF=0  angleLFb=0  angleLFc=0
      settings: AttributesFormatString=|
      | %<ID>
      | %<Vbase>V
      | %<VLF>pu
      | %<angleLF>deg.
      | %<Name>
  bus388 : powerlib/Measurements/Load Flow Bus  LConnTagsString=a  Phases=single  Connectors=on one side  ID=bus388  Vbase=400000  Vref=1  Vangle=0  VLF=1  VLFb=1  VLFc=1  angleLF=0  angleLFb=0  angleLFc=0
      settings: AttributesFormatString=|
      | %<ID>
      | %<Vbase>V
      | %<VLF>pu
      | %<angleLF>deg.
      | %<Name>
  bus389 : powerlib/Measurements/Load Flow Bus  LConnTagsString=a  Phases=single  Connectors=on one side  ID=bus389  Vbase=400000  Vref=1  Vangle=0  VLF=1  VLFb=1  VLFc=1  angleLF=0  angleLFb=0  angleLFc=0
      settings: AttributesFormatString=|
      | %<ID>
      | %<Vbase>V
      | %<VLF>pu
      | %<angleLF>deg.
      | %<Name>
  bus39 : powerlib/Measurements/Load Flow Bus  LConnTagsString=a  Phases=single  Connectors=on one side  ID=bus39  Vbase=400000  Vref=1  Vangle=0  VLF=1  VLFb=1  VLFc=1  angleLF=0  angleLFb=0  angleLFc=0
      settings: AttributesFormatString=|
      | %<ID>
      | %<Vbase>V
      | %<VLF>pu
      | %<angleLF>deg.
      | %<Name>
  bus390 : powerlib/Measurements/Load Flow Bus  LConnTagsString=a  Phases=single  Connectors=on one side  ID=bus390  Vbase=400000  Vref=1  Vangle=0  VLF=1  VLFb=1  VLFc=1  angleLF=0  angleLFb=0  angleLFc=0
      settings: AttributesFormatString=|
      | %<ID>
      | %<Vbase>V
      | %<VLF>pu
      | %<angleLF>deg.
      | %<Name>
  bus391 : powerlib/Measurements/Load Flow Bus  LConnTagsString=a  Phases=single  Connectors=on one side  ID=bus391  Vbase=400000  Vref=1  Vangle=0  VLF=1  VLFb=1  VLFc=1  angleLF=0  angleLFb=0  angleLFc=0
      settings: AttributesFormatString=|
      | %<ID>
      | %<Vbase>V
      | %<VLF>pu
      | %<angleLF>deg.
      | %<Name>
  bus392 : powerlib/Measurements/Load Flow Bus  LConnTagsString=a  Phases=single  Connectors=on one side  ID=bus392  Vbase=400000  Vref=1  Vangle=0  VLF=1  VLFb=1  VLFc=1  angleLF=0  angleLFb=0  angleLFc=0
      settings: AttributesFormatString=|
      | %<ID>
      | %<Vbase>V
      | %<VLF>pu
      | %<angleLF>deg.
      | %<Name>
  bus393 : powerlib/Measurements/Load Flow Bus  LConnTagsString=a  Phases=single  Connectors=on one side  ID=bus393  Vbase=400000  Vref=1  Vangle=0  VLF=1  VLFb=1  VLFc=1  angleLF=0  angleLFb=0  angleLFc=0
      settings: AttributesFormatString=|
      | %<ID>
      | %<Vbase>V
      | %<VLF>pu
      | %<angleLF>deg.
      | %<Name>
  bus394 : powerlib/Measurements/Load Flow Bus  LConnTagsString=a  Phases=single  Connectors=on one side  ID=bus394  Vbase=400000  Vref=1  Vangle=0  VLF=1  VLFb=1  VLFc=1  angleLF=0  angleLFb=0  angleLFc=0
      settings: AttributesFormatString=|
      | %<ID>
      | %<Vbase>V
      | %<VLF>pu
      | %<angleLF>deg.
      | %<Name>
  bus395 : powerlib/Measurements/Load Flow Bus  LConnTagsString=a  Phases=single  Connectors=on one side  ID=bus395  Vbase=400000  Vref=1  Vangle=0  VLF=1  VLFb=1  VLFc=1  angleLF=0  angleLFb=0  angleLFc=0
      settings: AttributesFormatString=|
      | %<ID>
      | %<Vbase>V
      | %<VLF>pu
      | %<angleLF>deg.
      | %<Name>
  bus396 : powerlib/Measurements/Load Flow Bus  LConnTagsString=a  Phases=single  Connectors=on one side  ID=bus396  Vbase=400000  Vref=1  Vangle=0  VLF=1  VLFb=1  VLFc=1  angleLF=0  angleLFb=0  angleLFc=0
      settings: AttributesFormatString=|
      | %<ID>
      | %<Vbase>V
      | %<VLF>pu
      | %<angleLF>deg.
      | %<Name>
  bus397 : powerlib/Measurements/Load Flow Bus  LConnTagsString=a  Phases=single  Connectors=on one side  ID=bus397  Vbase=400000  Vref=1  Vangle=0  VLF=1  VLFb=1  VLFc=1  angleLF=0  angleLFb=0  angleLFc=0
      settings: AttributesFormatString=|
      | %<ID>
      | %<Vbase>V
      | %<VLF>pu
      | %<angleLF>deg.
      | %<Name>
  bus398 : powerlib/Measurements/Load Flow Bus  LConnTagsString=a  Phases=single  Connectors=on one side  ID=bus398  Vbase=400000  Vref=1  Vangle=0  VLF=1  VLFb=1  VLFc=1  angleLF=0  angleLFb=0  angleLFc=0
      settings: AttributesFormatString=|
      | %<ID>
      | %<Vbase>V
      | %<VLF>pu
      | %<angleLF>deg.
      | %<Name>
  bus399 : powerlib/Measurements/Load Flow Bus  LConnTagsString=a  Phases=single  Connectors=on one side  ID=bus399  Vbase=400000  Vref=1  Vangle=0  VLF=1  VLFb=1  VLFc=1  angleLF=0  angleLFb=0  angleLFc=0
      settings: AttributesFormatString=|
      | %<ID>
      | %<Vbase>V
      | %<VLF>pu
      | %<angleLF>deg.
      | %<Name>
  bus4 : powerlib/Measurements/Load Flow Bus  LConnTagsString=a  Phases=single  Connectors=on one side  ID=bus4  Vbase=400000  Vref=1  Vangle=0  VLF=1  VLFb=1  VLFc=1  angleLF=0  angleLFb=0  angleLFc=0
      settings: AttributesFormatString=|
      | %<ID>
      | %<Vbase>V
      | %<VLF>pu
      | %<angleLF>deg.
      | %<Name>
  bus40 : powerlib/Measurements/Load Flow Bus  LConnTagsString=a  Phases=single  Connectors=on one side  ID=bus40  Vbase=400000  Vref=1  Vangle=0  VLF=1  VLFb=1  VLFc=1  angleLF=0  angleLFb=0  angleLFc=0
      settings: AttributesFormatString=|
      | %<ID>
      | %<Vbase>V
      | %<VLF>pu
      | %<angleLF>deg.
      | %<Name>
  bus400 : powerlib/Measurements/Load Flow Bus  LConnTagsString=a  Phases=single  Connectors=on one side  ID=bus400  Vbase=400000  Vref=1  Vangle=0  VLF=1  VLFb=1  VLFc=1  angleLF=0  angleLFb=0  angleLFc=0
      settings: AttributesFormatString=|
      | %<ID>
      | %<Vbase>V
      | %<VLF>pu
      | %<angleLF>deg.
      | %<Name>
  bus401 : powerlib/Measurements/Load Flow Bus  LConnTagsString=a  Phases=single  Connectors=on one side  ID=bus401  Vbase=400000  Vref=1  Vangle=0  VLF=1  VLFb=1  VLFc=1  angleLF=0  angleLFb=0  angleLFc=0
      settings: AttributesFormatString=|
      | %<ID>
      | %<Vbase>V
      | %<VLF>pu
      | %<angleLF>deg.
      | %<Name>
  bus402 : powerlib/Measurements/Load Flow Bus  LConnTagsString=a  Phases=single  Connectors=on one side  ID=bus402  Vbase=400000  Vref=1  Vangle=0  VLF=1  VLFb=1  VLFc=1  angleLF=0  angleLFb=0  angleLFc=0
      settings: AttributesFormatString=|
      | %<ID>
      | %<Vbase>V
      | %<VLF>pu
      | %<angleLF>deg.
      | %<Name>
  bus403 : powerlib/Measurements/Load Flow Bus  LConnTagsString=a  Phases=single  Connectors=on one side  ID=bus403  Vbase=400000  Vref=1  Vangle=0  VLF=1  VLFb=1  VLFc=1  angleLF=0  angleLFb=0  angleLFc=0
      settings: AttributesFormatString=|
      | %<ID>
      | %<Vbase>V
      | %<VLF>pu
      | %<angleLF>deg.
      | %<Name>
  bus404 : powerlib/Measurements/Load Flow Bus  LConnTagsString=a  Phases=single  Connectors=on one side  ID=bus404  Vbase=400000  Vref=1  Vangle=0  VLF=1  VLFb=1  VLFc=1  angleLF=0  angleLFb=0  angleLFc=0
      settings: AttributesFormatString=|
      | %<ID>
      | %<Vbase>V
      | %<VLF>pu
      | %<angleLF>deg.
      | %<Name>
  bus405 : powerlib/Measurements/Load Flow Bus  LConnTagsString=a  Phases=single  Connectors=on one side  ID=bus405  Vbase=400000  Vref=1  Vangle=0  VLF=1  VLFb=1  VLFc=1  angleLF=0  angleLFb=0  angleLFc=0
      settings: AttributesFormatString=|
      | %<ID>
      | %<Vbase>V
      | %<VLF>pu
      | %<angleLF>deg.
      | %<Name>
  bus406 : powerlib/Measurements/Load Flow Bus  LConnTagsString=a  Phases=single  Connectors=on one side  ID=bus406  Vbase=400000  Vref=1  Vangle=0  VLF=1  VLFb=1  VLFc=1  angleLF=0  angleLFb=0  angleLFc=0
      settings: AttributesFormatString=|
      | %<ID>
      | %<Vbase>V
      | %<VLF>pu
      | %<angleLF>deg.
      | %<Name>
  bus407 : powerlib/Measurements/Load Flow Bus  LConnTagsString=a  Phases=single  Connectors=on one side  ID=bus407  Vbase=400000  Vref=1  Vangle=0  VLF=1  VLFb=1  VLFc=1  angleLF=0  angleLFb=0  angleLFc=0
      settings: AttributesFormatString=|
      | %<ID>
      | %<Vbase>V
      | %<VLF>pu
      | %<angleLF>deg.
      | %<Name>
  bus408 : powerlib/Measurements/Load Flow Bus  LConnTagsString=a  Phases=single  Connectors=on one side  ID=bus408  Vbase=400000  Vref=1  Vangle=0  VLF=1  VLFb=1  VLFc=1  angleLF=0  angleLFb=0  angleLFc=0
      settings: AttributesFormatString=|
      | %<ID>
      | %<Vbase>V
      | %<VLF>pu
      | %<angleLF>deg.
      | %<Name>
  bus409 : powerlib/Measurements/Load Flow Bus  LConnTagsString=a  Phases=single  Connectors=on one side  ID=bus409  Vbase=400000  Vref=1  Vangle=0  VLF=1  VLFb=1  VLFc=1  angleLF=0  angleLFb=0  angleLFc=0
      settings: AttributesFormatString=|
      | %<ID>
      | %<Vbase>V
      | %<VLF>pu
      | %<angleLF>deg.
      | %<Name>
  bus41 : powerlib/Measurements/Load Flow Bus  LConnTagsString=a  Phases=single  Connectors=on one side  ID=bus41  Vbase=400000  Vref=1  Vangle=0  VLF=1  VLFb=1  VLFc=1  angleLF=0  angleLFb=0  angleLFc=0
      settings: AttributesFormatString=|
      | %<ID>
      | %<Vbase>V
      | %<VLF>pu
      | %<angleLF>deg.
      | %<Name>
  bus410 : powerlib/Measurements/Load Flow Bus  LConnTagsString=a  Phases=single  Connectors=on one side  ID=bus410  Vbase=400000  Vref=1  Vangle=0  VLF=1  VLFb=1  VLFc=1  angleLF=0  angleLFb=0  angleLFc=0
      settings: AttributesFormatString=|
      | %<ID>
      | %<Vbase>V
      | %<VLF>pu
      | %<angleLF>deg.
      | %<Name>
  bus411 : powerlib/Measurements/Load Flow Bus  LConnTagsString=a  Phases=single  Connectors=on one side  ID=bus411  Vbase=400000  Vref=1  Vangle=0  VLF=1  VLFb=1  VLFc=1  angleLF=0  angleLFb=0  angleLFc=0
      settings: AttributesFormatString=|
      | %<ID>
      | %<Vbase>V
      | %<VLF>pu
      | %<angleLF>deg.
      | %<Name>
  bus412 : powerlib/Measurements/Load Flow Bus  LConnTagsString=a  Phases=single  Connectors=on one side  ID=bus412  Vbase=400000  Vref=1  Vangle=0  VLF=1  VLFb=1  VLFc=1  angleLF=0  angleLFb=0  angleLFc=0
      settings: AttributesFormatString=|
      | %<ID>
      | %<Vbase>V
      | %<VLF>pu
      | %<angleLF>deg.
      | %<Name>
  bus413 : powerlib/Measurements/Load Flow Bus  LConnTagsString=a  Phases=single  Connectors=on one side  ID=bus413  Vbase=400000  Vref=1  Vangle=0  VLF=1  VLFb=1  VLFc=1  angleLF=0  angleLFb=0  angleLFc=0
      settings: AttributesFormatString=|
      | %<ID>
      | %<Vbase>V
      | %<VLF>pu
      | %<angleLF>deg.
      | %<Name>
  bus414 : powerlib/Measurements/Load Flow Bus  LConnTagsString=a  Phases=single  Connectors=on one side  ID=bus414  Vbase=400000  Vref=1  Vangle=0  VLF=1  VLFb=1  VLFc=1  angleLF=0  angleLFb=0  angleLFc=0
      settings: AttributesFormatString=|
      | %<ID>
      | %<Vbase>V
      | %<VLF>pu
      | %<angleLF>deg.
      | %<Name>
  bus415 : powerlib/Measurements/Load Flow Bus  LConnTagsString=a  Phases=single  Connectors=on one side  ID=bus415  Vbase=400000  Vref=1  Vangle=0  VLF=1  VLFb=1  VLFc=1  angleLF=0  angleLFb=0  angleLFc=0
      settings: AttributesFormatString=|
      | %<ID>
      | %<Vbase>V
      | %<VLF>pu
      | %<angleLF>deg.
      | %<Name>
  bus416 : powerlib/Measurements/Load Flow Bus  LConnTagsString=a  Phases=single  Connectors=on one side  ID=bus416  Vbase=400000  Vref=1  Vangle=0  VLF=1  VLFb=1  VLFc=1  angleLF=0  angleLFb=0  angleLFc=0
      settings: AttributesFormatString=|
      | %<ID>
      | %<Vbase>V
      | %<VLF>pu
      | %<angleLF>deg.
      | %<Name>
  bus417 : powerlib/Measurements/Load Flow Bus  LConnTagsString=a  Phases=single  Connectors=on one side  ID=bus417  Vbase=400000  Vref=1  Vangle=0  VLF=1  VLFb=1  VLFc=1  angleLF=0  angleLFb=0  angleLFc=0
      settings: AttributesFormatString=|
      | %<ID>
      | %<Vbase>V
      | %<VLF>pu
      | %<angleLF>deg.
      | %<Name>
  bus418 : powerlib/Measurements/Load Flow Bus  LConnTagsString=a  Phases=single  Connectors=on one side  ID=bus418  Vbase=400000  Vref=1  Vangle=0  VLF=1  VLFb=1  VLFc=1  angleLF=0  angleLFb=0  angleLFc=0
      settings: AttributesFormatString=|
      | %<ID>
      | %<Vbase>V
      | %<VLF>pu
      | %<angleLF>deg.
      | %<Name>
  bus419 : powerlib/Measurements/Load Flow Bus  LConnTagsString=a  Phases=single  Connectors=on one side  ID=bus419  Vbase=400000  Vref=1  Vangle=0  VLF=1  VLFb=1  VLFc=1  angleLF=0  angleLFb=0  angleLFc=0
      settings: AttributesFormatString=|
      | %<ID>
      | %<Vbase>V
      | %<VLF>pu
      | %<angleLF>deg.
      | %<Name>
  bus42 : powerlib/Measurements/Load Flow Bus  LConnTagsString=a  Phases=single  Connectors=on one side  ID=bus42  Vbase=400000  Vref=1  Vangle=0  VLF=1  VLFb=1  VLFc=1  angleLF=0  angleLFb=0  angleLFc=0
      settings: AttributesFormatString=|
      | %<ID>
      | %<Vbase>V
      | %<VLF>pu
      | %<angleLF>deg.
      | %<Name>
  bus43 : powerlib/Measurements/Load Flow Bus  LConnTagsString=a  Phases=single  Connectors=on one side  ID=bus43  Vbase=400000  Vref=1  Vangle=0  VLF=1  VLFb=1  VLFc=1  angleLF=0  angleLFb=0  angleLFc=0
      settings: AttributesFormatString=|
      | %<ID>
      | %<Vbase>V
      | %<VLF>pu
      | %<angleLF>deg.
      | %<Name>
  bus44 : powerlib/Measurements/Load Flow Bus  LConnTagsString=a  Phases=single  Connectors=on one side  ID=bus44  Vbase=400000  Vref=1  Vangle=0  VLF=1  VLFb=1  VLFc=1  angleLF=0  angleLFb=0  angleLFc=0
      settings: AttributesFormatString=|
      | %<ID>
      | %<Vbase>V
      | %<VLF>pu
      | %<angleLF>deg.
      | %<Name>
  bus45 : powerlib/Measurements/Load Flow Bus  LConnTagsString=a  Phases=single  Connectors=on one side  ID=bus45  Vbase=400000  Vref=1  Vangle=0  VLF=1  VLFb=1  VLFc=1  angleLF=0  angleLFb=0  angleLFc=0
      settings: AttributesFormatString=|
      | %<ID>
      | %<Vbase>V
      | %<VLF>pu
      | %<angleLF>deg.
      | %<Name>
  bus46 : powerlib/Measurements/Load Flow Bus  LConnTagsString=a  Phases=single  Connectors=on one side  ID=bus46  Vbase=400000  Vref=1  Vangle=0  VLF=1  VLFb=1  VLFc=1  angleLF=0  angleLFb=0  angleLFc=0
      settings: AttributesFormatString=|
      | %<ID>
      | %<Vbase>V
      | %<VLF>pu
      | %<angleLF>deg.
      | %<Name>
  bus47 : powerlib/Measurements/Load Flow Bus  LConnTagsString=a  Phases=single  Connectors=on one side  ID=bus47  Vbase=400000  Vref=1  Vangle=0  VLF=1  VLFb=1  VLFc=1  angleLF=0  angleLFb=0  angleLFc=0
      settings: AttributesFormatString=|
      | %<ID>
      | %<Vbase>V
      | %<VLF>pu
      | %<angleLF>deg.
      | %<Name>
  bus48 : powerlib/Measurements/Load Flow Bus  LConnTagsString=a  Phases=single  Connectors=on one side  ID=bus48  Vbase=400000  Vref=1  Vangle=0  VLF=1  VLFb=1  VLFc=1  angleLF=0  angleLFb=0  angleLFc=0
      settings: AttributesFormatString=|
      | %<ID>
      | %<Vbase>V
      | %<VLF>pu
      | %<angleLF>deg.
      | %<Name>
  bus49 : powerlib/Measurements/Load Flow Bus  LConnTagsString=a  Phases=single  Connectors=on one side  ID=bus49  Vbase=400000  Vref=1  Vangle=0  VLF=1  VLFb=1  VLFc=1  angleLF=0  angleLFb=0  angleLFc=0
      settings: AttributesFormatString=|
      | %<ID>
      | %<Vbase>V
      | %<VLF>pu
      | %<angleLF>deg.
      | %<Name>
  bus5 : powerlib/Measurements/Load Flow Bus  LConnTagsString=a  Phases=single  Connectors=on one side  ID=bus5  Vbase=400000  Vref=1  Vangle=0  VLF=1  VLFb=1  VLFc=1  angleLF=0  angleLFb=0  angleLFc=0
      settings: AttributesFormatString=|
      | %<ID>
      | %<Vbase>V
      | %<VLF>pu
      | %<angleLF>deg.
      | %<Name>
  bus50 : powerlib/Measurements/Load Flow Bus  LConnTagsString=a  Phases=single  Connectors=on one side  ID=bus50  Vbase=400000  Vref=1  Vangle=0  VLF=1  VLFb=1  VLFc=1  angleLF=0  angleLFb=0  angleLFc=0
      settings: AttributesFormatString=|
      | %<ID>
      | %<Vbase>V
      | %<VLF>pu
      | %<angleLF>deg.
      | %<Name>
  bus51 : powerlib/Measurements/Load Flow Bus  LConnTagsString=a  Phases=single  Connectors=on one side  ID=bus51  Vbase=400000  Vref=1  Vangle=0  VLF=1  VLFb=1  VLFc=1  angleLF=0  angleLFb=0  angleLFc=0
      settings: AttributesFormatString=|
      | %<ID>
      | %<Vbase>V
      | %<VLF>pu
      | %<angleLF>deg.
      | %<Name>
  bus52 : powerlib/Measurements/Load Flow Bus  LConnTagsString=a  Phases=single  Connectors=on one side  ID=bus52  Vbase=400000  Vref=1  Vangle=0  VLF=1  VLFb=1  VLFc=1  angleLF=0  angleLFb=0  angleLFc=0
      settings: AttributesFormatString=|
      | %<ID>
      | %<Vbase>V
      | %<VLF>pu
      | %<angleLF>deg.
      | %<Name>
  bus53 : powerlib/Measurements/Load Flow Bus  LConnTagsString=a  Phases=single  Connectors=on one side  ID=bus53  Vbase=400000  Vref=1  Vangle=0  VLF=1  VLFb=1  VLFc=1  angleLF=0  angleLFb=0  angleLFc=0
      settings: AttributesFormatString=|
      | %<ID>
      | %<Vbase>V
      | %<VLF>pu
      | %<angleLF>deg.
      | %<Name>
  bus54 : powerlib/Measurements/Load Flow Bus  LConnTagsString=a  Phases=single  Connectors=on one side  ID=bus54  Vbase=400000  Vref=1  Vangle=0  VLF=1  VLFb=1  VLFc=1  angleLF=0  angleLFb=0  angleLFc=0
      settings: AttributesFormatString=|
      | %<ID>
      | %<Vbase>V
      | %<VLF>pu
      | %<angleLF>deg.
      | %<Name>
  bus55 : powerlib/Measurements/Load Flow Bus  LConnTagsString=a  Phases=single  Connectors=on one side  ID=bus55  Vbase=400000  Vref=1  Vangle=0  VLF=1  VLFb=1  VLFc=1  angleLF=0  angleLFb=0  angleLFc=0
      settings: AttributesFormatString=|
      | %<ID>
      | %<Vbase>V
      | %<VLF>pu
      | %<angleLF>deg.
      | %<Name>
  bus56 : powerlib/Measurements/Load Flow Bus  LConnTagsString=a  Phases=single  Connectors=on one side  ID=bus56  Vbase=400000  Vref=1  Vangle=0  VLF=1  VLFb=1  VLFc=1  angleLF=0  angleLFb=0  angleLFc=0
      settings: AttributesFormatString=|
      | %<ID>
      | %<Vbase>V
      | %<VLF>pu
      | %<angleLF>deg.
      | %<Name>
  bus57 : powerlib/Measurements/Load Flow Bus  LConnTagsString=a  Phases=single  Connectors=on one side  ID=bus57  Vbase=400000  Vref=1  Vangle=0  VLF=1  VLFb=1  VLFc=1  angleLF=0  angleLFb=0  angleLFc=0
      settings: AttributesFormatString=|
      | %<ID>
      | %<Vbase>V
      | %<VLF>pu
      | %<angleLF>deg.
      | %<Name>
  bus58 : powerlib/Measurements/Load Flow Bus  LConnTagsString=a  Phases=single  Connectors=on one side  ID=bus58  Vbase=400000  Vref=1  Vangle=0  VLF=1  VLFb=1  VLFc=1  angleLF=0  angleLFb=0  angleLFc=0
      settings: AttributesFormatString=|
      | %<ID>
      | %<Vbase>V
      | %<VLF>pu
      | %<angleLF>deg.
      | %<Name>
  bus59 : powerlib/Measurements/Load Flow Bus  LConnTagsString=a  Phases=single  Connectors=on one side  ID=bus59  Vbase=400000  Vref=1  Vangle=0  VLF=1  VLFb=1  VLFc=1  angleLF=0  angleLFb=0  angleLFc=0
      settings: AttributesFormatString=|
      | %<ID>
      | %<Vbase>V
      | %<VLF>pu
      | %<angleLF>deg.
      | %<Name>
  bus6 : powerlib/Measurements/Load Flow Bus  LConnTagsString=a  Phases=single  Connectors=on one side  ID=bus6  Vbase=400000  Vref=1  Vangle=0  VLF=1  VLFb=1  VLFc=1  angleLF=0  angleLFb=0  angleLFc=0
      settings: AttributesFormatString=|
      | %<ID>
      | %<Vbase>V
      | %<VLF>pu
      | %<angleLF>deg.
      | %<Name>
  bus60 : powerlib/Measurements/Load Flow Bus  LConnTagsString=a  Phases=single  Connectors=on one side  ID=bus60  Vbase=400000  Vref=1  Vangle=0  VLF=1  VLFb=1  VLFc=1  angleLF=0  angleLFb=0  angleLFc=0
      settings: AttributesFormatString=|
      | %<ID>
      | %<Vbase>V
      | %<VLF>pu
      | %<angleLF>deg.
      | %<Name>
  bus61 : powerlib/Measurements/Load Flow Bus  LConnTagsString=a  Phases=single  Connectors=on one side  ID=bus61  Vbase=400000  Vref=1  Vangle=0  VLF=1  VLFb=1  VLFc=1  angleLF=0  angleLFb=0  angleLFc=0
      settings: AttributesFormatString=|
      | %<ID>
      | %<Vbase>V
      | %<VLF>pu
      | %<angleLF>deg.
      | %<Name>
  bus62 : powerlib/Measurements/Load Flow Bus  LConnTagsString=a  Phases=single  Connectors=on one side  ID=bus62  Vbase=400000  Vref=1  Vangle=0  VLF=1  VLFb=1  VLFc=1  angleLF=0  angleLFb=0  angleLFc=0
      settings: AttributesFormatString=|
      | %<ID>
      | %<Vbase>V
      | %<VLF>pu
      | %<angleLF>deg.
      | %<Name>
  bus63 : powerlib/Measurements/Load Flow Bus  LConnTagsString=a  Phases=single  Connectors=on one side  ID=bus63  Vbase=400000  Vref=1  Vangle=0  VLF=1  VLFb=1  VLFc=1  angleLF=0  angleLFb=0  angleLFc=0
      settings: AttributesFormatString=|
      | %<ID>
      | %<Vbase>V
      | %<VLF>pu
      | %<angleLF>deg.
      | %<Name>
  bus64 : powerlib/Measurements/Load Flow Bus  LConnTagsString=a  Phases=single  Connectors=on one side  ID=bus64  Vbase=400000  Vref=1  Vangle=0  VLF=1  VLFb=1  VLFc=1  angleLF=0  angleLFb=0  angleLFc=0
      settings: AttributesFormatString=|
      | %<ID>
      | %<Vbase>V
      | %<VLF>pu
      | %<angleLF>deg.
      | %<Name>
  bus65 : powerlib/Measurements/Load Flow Bus  LConnTagsString=a  Phases=single  Connectors=on one side  ID=bus65  Vbase=400000  Vref=1  Vangle=0  VLF=1  VLFb=1  VLFc=1  angleLF=0  angleLFb=0  angleLFc=0
      settings: AttributesFormatString=|
      | %<ID>
      | %<Vbase>V
      | %<VLF>pu
      | %<angleLF>deg.
      | %<Name>
  bus66 : powerlib/Measurements/Load Flow Bus  LConnTagsString=a  Phases=single  Connectors=on one side  ID=bus66  Vbase=400000  Vref=1  Vangle=0  VLF=1  VLFb=1  VLFc=1  angleLF=0  angleLFb=0  angleLFc=0
      settings: AttributesFormatString=|
      | %<ID>
      | %<Vbase>V
      | %<VLF>pu
      | %<angleLF>deg.
      | %<Name>
  bus67 : powerlib/Measurements/Load Flow Bus  LConnTagsString=a  Phases=single  Connectors=on one side  ID=bus67  Vbase=400000  Vref=1  Vangle=0  VLF=1  VLFb=1  VLFc=1  angleLF=0  angleLFb=0  angleLFc=0
      settings: AttributesFormatString=|
      | %<ID>
      | %<Vbase>V
      | %<VLF>pu
      | %<angleLF>deg.
      | %<Name>
  bus68 : powerlib/Measurements/Load Flow Bus  LConnTagsString=a  Phases=single  Connectors=on one side  ID=bus68  Vbase=400000  Vref=1  Vangle=0  VLF=1  VLFb=1  VLFc=1  angleLF=0  angleLFb=0  angleLFc=0
      settings: AttributesFormatString=|
      | %<ID>
      | %<Vbase>V
      | %<VLF>pu
      | %<angleLF>deg.
      | %<Name>
  bus69 : powerlib/Measurements/Load Flow Bus  LConnTagsString=a  Phases=single  Connectors=on one side  ID=bus69  Vbase=400000  Vref=1  Vangle=0  VLF=1  VLFb=1  VLFc=1  angleLF=0  angleLFb=0  angleLFc=0
      settings: AttributesFormatString=|
      | %<ID>
      | %<Vbase>V
      | %<VLF>pu
      | %<angleLF>deg.
      | %<Name>
  bus7 : powerlib/Measurements/Load Flow Bus  LConnTagsString=a  Phases=single  Connectors=on one side  ID=bus7  Vbase=400000  Vref=1  Vangle=0  VLF=1  VLFb=1  VLFc=1  angleLF=0  angleLFb=0  angleLFc=0
      settings: AttributesFormatString=|
      | %<ID>
      | %<Vbase>V
      | %<VLF>pu
      | %<angleLF>deg.
      | %<Name>
  bus70 : powerlib/Measurements/Load Flow Bus  LConnTagsString=a  Phases=single  Connectors=on one side  ID=bus70  Vbase=400000  Vref=1  Vangle=0  VLF=1  VLFb=1  VLFc=1  angleLF=0  angleLFb=0  angleLFc=0
      settings: AttributesFormatString=|
      | %<ID>
      | %<Vbase>V
      | %<VLF>pu
      | %<angleLF>deg.
      | %<Name>
  bus71 : powerlib/Measurements/Load Flow Bus  LConnTagsString=a  Phases=single  Connectors=on one side  ID=bus71  Vbase=400000  Vref=1  Vangle=0  VLF=1  VLFb=1  VLFc=1  angleLF=0  angleLFb=0  angleLFc=0
      settings: AttributesFormatString=|
      | %<ID>
      | %<Vbase>V
      | %<VLF>pu
      | %<angleLF>deg.
      | %<Name>
  bus72 : powerlib/Measurements/Load Flow Bus  LConnTagsString=a  Phases=single  Connectors=on one side  ID=bus72  Vbase=400000  Vref=1  Vangle=0  VLF=1  VLFb=1  VLFc=1  angleLF=0  angleLFb=0  angleLFc=0
      settings: AttributesFormatString=|
      | %<ID>
      | %<Vbase>V
      | %<VLF>pu
      | %<angleLF>deg.
      | %<Name>
  bus73 : powerlib/Measurements/Load Flow Bus  LConnTagsString=a  Phases=single  Connectors=on one side  ID=bus73  Vbase=400000  Vref=1  Vangle=0  VLF=1  VLFb=1  VLFc=1  angleLF=0  angleLFb=0  angleLFc=0
      settings: AttributesFormatString=|
      | %<ID>
      | %<Vbase>V
      | %<VLF>pu
      | %<angleLF>deg.
      | %<Name>
  bus74 : powerlib/Measurements/Load Flow Bus  LConnTagsString=a  Phases=single  Connectors=on one side  ID=bus74  Vbase=400000  Vref=1  Vangle=0  VLF=1  VLFb=1  VLFc=1  angleLF=0  angleLFb=0  angleLFc=0
      settings: AttributesFormatString=|
      | %<ID>
      | %<Vbase>V
      | %<VLF>pu
      | %<angleLF>deg.
      | %<Name>
  bus75 : powerlib/Measurements/Load Flow Bus  LConnTagsString=a  Phases=single  Connectors=on one side  ID=bus75  Vbase=400000  Vref=1  Vangle=0  VLF=1  VLFb=1  VLFc=1  angleLF=0  angleLFb=0  angleLFc=0
      settings: AttributesFormatString=|
      | %<ID>
      | %<Vbase>V
      | %<VLF>pu
      | %<angleLF>deg.
      | %<Name>
  bus76 : powerlib/Measurements/Load Flow Bus  LConnTagsString=a  Phases=single  Connectors=on one side  ID=bus76  Vbase=400000  Vref=1  Vangle=0  VLF=1  VLFb=1  VLFc=1  angleLF=0  angleLFb=0  angleLFc=0
      settings: AttributesFormatString=|
      | %<ID>
      | %<Vbase>V
      | %<VLF>pu
      | %<angleLF>deg.
      | %<Name>
  bus77 : powerlib/Measurements/Load Flow Bus  LConnTagsString=a  Phases=single  Connectors=on one side  ID=bus77  Vbase=400000  Vref=1  Vangle=0  VLF=1  VLFb=1  VLFc=1  angleLF=0  angleLFb=0  angleLFc=0
      settings: AttributesFormatString=|
      | %<ID>
      | %<Vbase>V
      | %<VLF>pu
      | %<angleLF>deg.
      | %<Name>
  bus78 : powerlib/Measurements/Load Flow Bus  LConnTagsString=a  Phases=single  Connectors=on one side  ID=bus78  Vbase=400000  Vref=1  Vangle=0  VLF=1  VLFb=1  VLFc=1  angleLF=0  angleLFb=0  angleLFc=0
      settings: AttributesFormatString=|
      | %<ID>
      | %<Vbase>V
      | %<VLF>pu
      | %<angleLF>deg.
      | %<Name>
  bus79 : powerlib/Measurements/Load Flow Bus  LConnTagsString=a  Phases=single  Connectors=on one side  ID=bus79  Vbase=400000  Vref=1  Vangle=0  VLF=1  VLFb=1  VLFc=1  angleLF=0  angleLFb=0  angleLFc=0
      settings: AttributesFormatString=|
      | %<ID>
      | %<Vbase>V
      | %<VLF>pu
      | %<angleLF>deg.
      | %<Name>
  bus8 : powerlib/Measurements/Load Flow Bus  LConnTagsString=a  Phases=single  Connectors=on one side  ID=bus8  Vbase=400000  Vref=1  Vangle=0  VLF=1  VLFb=1  VLFc=1  angleLF=0  angleLFb=0  angleLFc=0
      settings: AttributesFormatString=|
      | %<ID>
      | %<Vbase>V
      | %<VLF>pu
      | %<angleLF>deg.
      | %<Name>
  bus80 : powerlib/Measurements/Load Flow Bus  LConnTagsString=a  Phases=single  Connectors=on one side  ID=bus80  Vbase=400000  Vref=1  Vangle=0  VLF=1  VLFb=1  VLFc=1  angleLF=0  angleLFb=0  angleLFc=0
      settings: AttributesFormatString=|
      | %<ID>
      | %<Vbase>V
      | %<VLF>pu
      | %<angleLF>deg.
      | %<Name>
  bus81 : powerlib/Measurements/Load Flow Bus  LConnTagsString=a  Phases=single  Connectors=on one side  ID=bus81  Vbase=400000  Vref=1  Vangle=0  VLF=1  VLFb=1  VLFc=1  angleLF=0  angleLFb=0  angleLFc=0
      settings: AttributesFormatString=|
      | %<ID>
      | %<Vbase>V
      | %<VLF>pu
      | %<angleLF>deg.
      | %<Name>
  bus82 : powerlib/Measurements/Load Flow Bus  LConnTagsString=a  Phases=single  Connectors=on one side  ID=bus82  Vbase=400000  Vref=1  Vangle=0  VLF=1  VLFb=1  VLFc=1  angleLF=0  angleLFb=0  angleLFc=0
      settings: AttributesFormatString=|
      | %<ID>
      | %<Vbase>V
      | %<VLF>pu
      | %<angleLF>deg.
      | %<Name>
  bus83 : powerlib/Measurements/Load Flow Bus  LConnTagsString=a  Phases=single  Connectors=on one side  ID=bus83  Vbase=400000  Vref=1  Vangle=0  VLF=1  VLFb=1  VLFc=1  angleLF=0  angleLFb=0  angleLFc=0
      settings: AttributesFormatString=|
      | %<ID>
      | %<Vbase>V
      | %<VLF>pu
      | %<angleLF>deg.
      | %<Name>
  bus84 : powerlib/Measurements/Load Flow Bus  LConnTagsString=a  Phases=single  Connectors=on one side  ID=bus84  Vbase=400000  Vref=1  Vangle=0  VLF=1  VLFb=1  VLFc=1  angleLF=0  angleLFb=0  angleLFc=0
      settings: AttributesFormatString=|
      | %<ID>
      | %<Vbase>V
      | %<VLF>pu
      | %<angleLF>deg.
      | %<Name>
  bus85 : powerlib/Measurements/Load Flow Bus  LConnTagsString=a  Phases=single  Connectors=on one side  ID=bus85  Vbase=400000  Vref=1  Vangle=0  VLF=1  VLFb=1  VLFc=1  angleLF=0  angleLFb=0  angleLFc=0
      settings: AttributesFormatString=|
      | %<ID>
      | %<Vbase>V
      | %<VLF>pu
      | %<angleLF>deg.
      | %<Name>
  bus86 : powerlib/Measurements/Load Flow Bus  LConnTagsString=a  Phases=single  Connectors=on one side  ID=bus86  Vbase=400000  Vref=1  Vangle=0  VLF=1  VLFb=1  VLFc=1  angleLF=0  angleLFb=0  angleLFc=0
      settings: AttributesFormatString=|
      | %<ID>
      | %<Vbase>V
      | %<VLF>pu
      | %<angleLF>deg.
      | %<Name>
  bus87 : powerlib/Measurements/Load Flow Bus  LConnTagsString=a  Phases=single  Connectors=on one side  ID=bus87  Vbase=400000  Vref=1  Vangle=0  VLF=1  VLFb=1  VLFc=1  angleLF=0  angleLFb=0  angleLFc=0
      settings: AttributesFormatString=|
      | %<ID>
      | %<Vbase>V
      | %<VLF>pu
      | %<angleLF>deg.
      | %<Name>
  bus88 : powerlib/Measurements/Load Flow Bus  LConnTagsString=a  Phases=single  Connectors=on one side  ID=bus88  Vbase=400000  Vref=1  Vangle=0  VLF=1  VLFb=1  VLFc=1  angleLF=0  angleLFb=0  angleLFc=0
      settings: AttributesFormatString=|
      | %<ID>
      | %<Vbase>V
      | %<VLF>pu
      | %<angleLF>deg.
      | %<Name>
  bus89 : powerlib/Measurements/Load Flow Bus  LConnTagsString=a  Phases=single  Connectors=on one side  ID=bus89  Vbase=400000  Vref=1  Vangle=0  VLF=1  VLFb=1  VLFc=1  angleLF=0  angleLFb=0  angleLFc=0
      settings: AttributesFormatString=|
      | %<ID>
      | %<Vbase>V
      | %<VLF>pu
      | %<angleLF>deg.
      | %<Name>
  bus9 : powerlib/Measurements/Load Flow Bus  LConnTagsString=a  Phases=single  Connectors=on one side  ID=bus9  Vbase=400000  Vref=1  Vangle=0  VLF=1  VLFb=1  VLFc=1  angleLF=0  angleLFb=0  angleLFc=0
      settings: AttributesFormatString=|
      | %<ID>
      | %<Vbase>V
      | %<VLF>pu
      | %<angleLF>deg.
      | %<Name>
  bus90 : powerlib/Measurements/Load Flow Bus  LConnTagsString=a  Phases=single  Connectors=on one side  ID=bus90  Vbase=400000  Vref=1  Vangle=0  VLF=1  VLFb=1  VLFc=1  angleLF=0  angleLFb=0  angleLFc=0
      settings: AttributesFormatString=|
      | %<ID>
      | %<Vbase>V
      | %<VLF>pu
      | %<angleLF>deg.
      | %<Name>
  bus91 : powerlib/Measurements/Load Flow Bus  LConnTagsString=a  Phases=single  Connectors=on one side  ID=bus91  Vbase=400000  Vref=1  Vangle=0  VLF=1  VLFb=1  VLFc=1  angleLF=0  angleLFb=0  angleLFc=0
      settings: AttributesFormatString=|
      | %<ID>
      | %<Vbase>V
      | %<VLF>pu
      | %<angleLF>deg.
      | %<Name>
  bus92 : powerlib/Measurements/Load Flow Bus  LConnTagsString=a  Phases=single  Connectors=on one side  ID=bus92  Vbase=400000  Vref=1  Vangle=0  VLF=1  VLFb=1  VLFc=1  angleLF=0  angleLFb=0  angleLFc=0
      settings: AttributesFormatString=|
      | %<ID>
      | %<Vbase>V
      | %<VLF>pu
      | %<angleLF>deg.
      | %<Name>
  bus93 : powerlib/Measurements/Load Flow Bus  LConnTagsString=a  Phases=single  Connectors=on one side  ID=bus93  Vbase=400000  Vref=1  Vangle=0  VLF=1  VLFb=1  VLFc=1  angleLF=0  angleLFb=0  angleLFc=0
      settings: AttributesFormatString=|
      | %<ID>
      | %<Vbase>V
      | %<VLF>pu
      | %<angleLF>deg.
      | %<Name>
  bus94 : powerlib/Measurements/Load Flow Bus  LConnTagsString=a  Phases=single  Connectors=on one side  ID=bus94  Vbase=400000  Vref=1  Vangle=0  VLF=1  VLFb=1  VLFc=1  angleLF=0  angleLFb=0  angleLFc=0
      settings: AttributesFormatString=|
      | %<ID>
      | %<Vbase>V
      | %<VLF>pu
      | %<angleLF>deg.
      | %<Name>
  bus95 : powerlib/Measurements/Load Flow Bus  LConnTagsString=a  Phases=single  Connectors=on one side  ID=bus95  Vbase=400000  Vref=1  Vangle=0  VLF=1  VLFb=1  VLFc=1  angleLF=0  angleLFb=0  angleLFc=0
      settings: AttributesFormatString=|
      | %<ID>
      | %<Vbase>V
      | %<VLF>pu
      | %<angleLF>deg.
      | %<Name>
  bus96 : powerlib/Measurements/Load Flow Bus  LConnTagsString=a  Phases=single  Connectors=on one side  ID=bus96  Vbase=400000  Vref=1  Vangle=0  VLF=1  VLFb=1  VLFc=1  angleLF=0  angleLFb=0  angleLFc=0
      settings: AttributesFormatString=|
      | %<ID>
      | %<Vbase>V
      | %<VLF>pu
      | %<angleLF>deg.
      | %<Name>
  bus97 : powerlib/Measurements/Load Flow Bus  LConnTagsString=a  Phases=single  Connectors=on one side  ID=bus97  Vbase=400000  Vref=1  Vangle=0  VLF=1  VLFb=1  VLFc=1  angleLF=0  angleLFb=0  angleLFc=0
      settings: AttributesFormatString=|
      | %<ID>
      | %<Vbase>V
      | %<VLF>pu
      | %<angleLF>deg.
      | %<Name>
  bus98 : powerlib/Measurements/Load Flow Bus  LConnTagsString=a  Phases=single  Connectors=on one side  ID=bus98  Vbase=400000  Vref=1  Vangle=0  VLF=1  VLFb=1  VLFc=1  angleLF=0  angleLFb=0  angleLFc=0
      settings: AttributesFormatString=|
      | %<ID>
      | %<Vbase>V
      | %<VLF>pu
      | %<angleLF>deg.
      | %<Name>
  bus99 : powerlib/Measurements/Load Flow Bus  LConnTagsString=a  Phases=single  Connectors=on one side  ID=bus99  Vbase=400000  Vref=1  Vangle=0  VLF=1  VLFb=1  VLFc=1  angleLF=0  angleLFb=0  angleLFc=0
      settings: AttributesFormatString=|
      | %<ID>
      | %<Vbase>V
      | %<VLF>pu
      | %<angleLF>deg.
      | %<Name>
  powergui : powerlib/powergui  Priority=1  SimulationMode=Phasor  SolverType=Tustin/Backward Euler (TBE)  SampleTime=50e-6  frequency=50  SPID=off  DisableSnubberDevices=off  DisableRonSwitches=off  DisableVfSwitches=off  SwTol=0  DisplayEquations=off  Interpol=off  ExternalGateDelay=off  methode=off  Ts=10  FunctionMessages=off  echomessages=off  HookPort=off  EnableUseOfTLC=off  x0status=blocks  frequencyindice=50  Pbase=3000e6  ErrMax=0.0001  Iterations=50  UnitsV=V  UnitsW=W  buscounter=0  RestoreLinks=warning  ResistiveCurrentMeasurement=off  Frange=[0:2:500]  Ylog=off  Xlog=on  ShowGrid=off  save=off  variable=ZData  structure=0  ZoomFFT=off  StartTime=0.0  cycles=1  DisplayStyle=1  fundamental=60  FreqAxis=off  MaxFrequency=1000  frequencyindicesteady=1  RmsSteady=1  display=off
  connections:
  _CN_143861248_400000_CN_95749833_400000/LConn1 -- T_143861248_400000_Pembroke_Substation/LConn1 -- _CN_143861248_400000_CN_95896505_400000/LConn1 -- _CN_143861248_400000_CN_95895489_400000/LConn1 -- _CN_143861248_400000_CN_192220229_400000/LConn1 -- _CN_143861248_400000_CN_95600440_400000/LConn1
  _CN_143861248_400000_CN_95749833_400000/LConn2 -- T_143861248_400000_Pembroke_Substation/LConn2 -- _CN_143861248_400000_CN_95896505_400000/LConn2 -- _CN_143861248_400000_CN_95895489_400000/LConn2 -- _CN_143861248_400000_CN_192220229_400000/LConn2 -- _CN_143861248_400000_CN_95600440_400000/LConn2
  _CN_143861248_400000_CN_95749833_400000/LConn3 -- T_143861248_400000_Pembroke_Substation/LConn3 -- _CN_143861248_400000_CN_95896505_400000/LConn3 -- _CN_143861248_400000_CN_95895489_400000/LConn3 -- _CN_143861248_400000_CN_192220229_400000/LConn3 -- _CN_143861248_400000_CN_95600440_400000/LConn3 -- bus1/LConn1
  _CN_143861248_400000_CN_95749833_400000/RConn1 -- T_95749833_400000;275000_CILF_Cilfynydd/LConn1 -- _CN_42799627_400000_CN_95749833_400000/LConn1
  _CN_143861248_400000_CN_95749833_400000/RConn2 -- T_95749833_400000;275000_CILF_Cilfynydd/LConn2 -- _CN_42799627_400000_CN_95749833_400000/LConn2
  _CN_143861248_400000_CN_95749833_400000/RConn3 -- T_95749833_400000;275000_CILF_Cilfynydd/LConn3 -- _CN_42799627_400000_CN_95749833_400000/LConn3 -- bus2/LConn1
  _CN_143861248_400000_CN_95896505_400000/RConn1 -- T_95896505__/LConn1 -- _CN_92483460_400000_CN_95896505_400000/LConn1
  _CN_143861248_400000_CN_95896505_400000/RConn2 -- T_95896505__/LConn2 -- _CN_92483460_400000_CN_95896505_400000/LConn2
  _CN_143861248_400000_CN_95896505_400000/RConn3 -- T_95896505__/LConn3 -- _CN_92483460_400000_CN_95896505_400000/LConn3 -- bus3/LConn1
  T_95895489_400000_/LConn1 -- _CN_143861248_400000_CN_95895489_400000/RConn1
  T_95895489_400000_/LConn2 -- _CN_143861248_400000_CN_95895489_400000/RConn2
  _CN_143861248_400000_CN_95895489_400000/RConn3 -- T_95895489_400000_/LConn3 -- bus4/LConn1
  T_192220229_400000_Swansea_North_Substation/LConn1 -- _CN_143861248_400000_CN_192220229_400000/RConn1
  T_192220229_400000_Swansea_North_Substation/LConn2 -- _CN_143861248_400000_CN_192220229_400000/RConn2
  _CN_143861248_400000_CN_192220229_400000/RConn3 -- T_192220229_400000_Swansea_North_Substation/LConn3 -- bus5/LConn1
  T_95600440_400000_Swansea_North_Substation/LConn1 -- _CN_143861248_400000_CN_95600440_400000/RConn1
  T_95600440_400000_Swansea_North_Substation/LConn2 -- _CN_143861248_400000_CN_95600440_400000/RConn2
  _CN_143861248_400000_CN_95600440_400000/RConn3 -- T_95600440_400000_Swansea_North_Substation/LConn3 -- bus6/LConn1
  National_Grid_Cowley_Seven_Springs_CN_51424257_400000_CN_23059230_400000/LConn1 -- T_51424257__Hinksey_South___Cable_Sealing_End_Compound/LConn1 -- _CN_51424257_400000_CN_32117744_400000/LConn1
  National_Grid_Cowley_Seven_Springs_CN_51424257_400000_CN_23059230_400000/LConn2 -- T_51424257__Hinksey_South___Cable_Sealing_End_Compound/LConn2 -- _CN_51424257_400000_CN_32117744_400000/LConn2
  National_Grid_Cowley_Seven_Springs_CN_51424257_400000_CN_23059230_400000/LConn3 -- T_51424257__Hinksey_South___Cable_Sealing_End_Compound/LConn3 -- _CN_51424257_400000_CN_32117744_400000/LConn3 -- bus7/LConn1
  National_Grid_Cowley_Seven_Springs_CN_51424257_400000_CN_23059230_400000/RConn1 -- T_23059230_400000;132000_Cowley_Substation/LConn1 -- _CN_23059230_400000_CN_30904448_400000/LConn1 -- _CN_23059230_400000_CN_92340133_400000/LConn1 -- _CN_23059230_400000_CN_89453364_400000/LConn1
  National_Grid_Cowley_Seven_Springs_CN_51424257_400000_CN_23059230_400000/RConn2 -- T_23059230_400000;132000_Cowley_Substation/LConn2 -- _CN_23059230_400000_CN_30904448_400000/LConn2 -- _CN_23059230_400000_CN_92340133_400000/LConn2 -- _CN_23059230_400000_CN_89453364_400000/LConn2
  National_Grid_Cowley_Seven_Springs_CN_51424257_400000_CN_23059230_400000/RConn3 -- T_23059230_400000;132000_Cowley_Substation/LConn3 -- _CN_23059230_400000_CN_30904448_400000/LConn3 -- _CN_23059230_400000_CN_92340133_400000/LConn3 -- _CN_23059230_400000_CN_89453364_400000/LConn3 -- bus8/LConn1
  _CN_51424257_400000_CN_32117744_400000/RConn1 -- T_32117744__Hinksey_North___Cable_Sealing_End_Compound/LConn1 -- _CN_95279334_400000_CN_32117744_400000/LConn1
  _CN_51424257_400000_CN_32117744_400000/RConn2 -- T_32117744__Hinksey_North___Cable_Sealing_End_Compound/LConn2 -- _CN_95279334_400000_CN_32117744_400000/LConn2
  _CN_51424257_400000_CN_32117744_400000/RConn3 -- T_32117744__Hinksey_North___Cable_Sealing_End_Compound/LConn3 -- _CN_95279334_400000_CN_32117744_400000/LConn3 -- bus9/LConn1
  T_376450057_400000_/LConn1 -- _CN_376450057_400000_CN_143902275_400000/LConn1
  T_376450057_400000_/LConn2 -- _CN_376450057_400000_CN_143902275_400000/LConn2
  _CN_376450057_400000_CN_143902275_400000/LConn3 -- T_376450057_400000_/LConn3 -- bus10/LConn1
  _CN_376450057_400000_CN_143902275_400000/RConn1 -- G_143902275_Spalding_Power_Station/RConn1 -- _CN_38528291_400000_CN_143902275_400000/LConn1
  _CN_376450057_400000_CN_143902275_400000/RConn2 -- G_143902275_Spalding_Power_Station/RConn2 -- _CN_38528291_400000_CN_143902275_400000/LConn2
  _CN_376450057_400000_CN_143902275_400000/RConn3 -- G_143902275_Spalding_Power_Station/RConn3 -- _CN_38528291_400000_CN_143902275_400000/LConn3 -- bus11/LConn1
  _CN_42799627_400000_CN_375637875_400000/LConn1 -- T_42799627__Cable_tunnel_shaft/LConn1 -- Cable_tunnel_CN_42799627_400000_CN_103962437_400000/LConn1 -- _CN_42799627_400000_CN_42800878_400000/LConn1 -- _CN_42799627_400000_CN_95749833_400000/RConn1
  _CN_42799627_400000_CN_375637875_400000/LConn2 -- T_42799627__Cable_tunnel_shaft/LConn2 -- Cable_tunnel_CN_42799627_400000_CN_103962437_400000/LConn2 -- _CN_42799627_400000_CN_42800878_400000/LConn2 -- _CN_42799627_400000_CN_95749833_400000/RConn2
  _CN_42799627_400000_CN_375637875_400000/LConn3 -- T_42799627__Cable_tunnel_shaft/LConn3 -- Cable_tunnel_CN_42799627_400000_CN_103962437_400000/LConn3 -- bus12/LConn1 -- _CN_42799627_400000_CN_42800878_400000/LConn3 -- _CN_42799627_400000_CN_95749833_400000/RConn3
  T_375637875_400000;275000_WHSO_Whitson/LConn1 -- _CN_42799627_400000_CN_375637875_400000/RConn1
  T_375637875_400000;275000_WHSO_Whitson/LConn2 -- _CN_42799627_400000_CN_375637875_400000/RConn2
  _CN_42799627_400000_CN_375637875_400000/RConn3 -- T_375637875_400000;275000_WHSO_Whitson/LConn3 -- bus13/LConn1
  T_42800878_400000_IMPP_Imperial_Park/LConn1 -- _CN_42799627_400000_CN_42800878_400000/RConn1
  T_42800878_400000_IMPP_Imperial_Park/LConn2 -- _CN_42799627_400000_CN_42800878_400000/RConn2
  _CN_42799627_400000_CN_42800878_400000/RConn3 -- T_42800878_400000_IMPP_Imperial_Park/LConn3 -- bus14/LConn1
  Cable_tunnel_CN_42799627_400000_CN_103962437_400000/RConn1 -- T_103962437__Cable_tunnel_shaft/LConn1 -- National_Grid_Melksham_?_CN_103915328_400000_CN_103962437_400000/LConn1
  Cable_tunnel_CN_42799627_400000_CN_103962437_400000/RConn2 -- T_103962437__Cable_tunnel_shaft/LConn2 -- National_Grid_Melksham_?_CN_103915328_400000_CN_103962437_400000/LConn2
  Cable_tunnel_CN_42799627_400000_CN_103962437_400000/RConn3 -- T_103962437__Cable_tunnel_shaft/LConn3 -- National_Grid_Melksham_?_CN_103915328_400000_CN_103962437_400000/LConn3 -- bus15/LConn1
  _CN_143384076_400000_CN_143383456_400000/LConn1 -- T_143384076_400000_Strathaven_Substation/LConn1 -- SP_Transmission_Coalburn_?_CN_143384076_400000_CN_96905262_400000/LConn1 -- SP_Transmission_Coalburn_?_CN_143384076_400000_CN_262532045_400000/LConn1 -- SP_Transmission_Coalburn_?_CN_143384076_400000_CN_262523325_400000/LConn1 -- SP_Transmission_Coalburn_?_CN_143384076_400000_CN_97551518_400000/LConn1 -- _CN_143384076_400000_CN_284874050_400000/LConn1 -- _CN_143384076_400000_CN_100077745_400000/LConn1 -- _CN_143384076_400000_CN_308653841_400000/LConn1 -- _CN_143384076_400000_CN_86071326_400000/LConn1 -- _CN_143384076_400000_CN_91038272_400000/LConn1 -- _CN_143384076_400000_CN_143398452_400000/LConn1 -- _CN_143384076_400000_CN_308653843_400000/LConn1
  _CN_143384076_400000_CN_143383456_400000/LConn2 -- T_143384076_400000_Strathaven_Substation/LConn2 -- SP_Transmission_Coalburn_?_CN_143384076_400000_CN_96905262_400000/LConn2 -- SP_Transmission_Coalburn_?_CN_143384076_400000_CN_262532045_400000/LConn2 -- SP_Transmission_Coalburn_?_CN_143384076_400000_CN_262523325_400000/LConn2 -- SP_Transmission_Coalburn_?_CN_143384076_400000_CN_97551518_400000/LConn2 -- _CN_143384076_400000_CN_284874050_400000/LConn2 -- _CN_143384076_400000_CN_100077745_400000/LConn2 -- _CN_143384076_400000_CN_308653841_400000/LConn2 -- _CN_143384076_400000_CN_86071326_400000/LConn2 -- _CN_143384076_400000_CN_91038272_400000/LConn2 -- _CN_143384076_400000_CN_143398452_400000/LConn2 -- _CN_143384076_400000_CN_308653843_400000/LConn2
  _CN_143384076_400000_CN_143383456_400000/LConn3 -- T_143384076_400000_Strathaven_Substation/LConn3 -- SP_Transmission_Coalburn_?_CN_143384076_400000_CN_96905262_400000/LConn3 -- SP_Transmission_Coalburn_?_CN_143384076_400000_CN_262532045_400000/LConn3 -- SP_Transmission_Coalburn_?_CN_143384076_400000_CN_262523325_400000/LConn3 -- SP_Transmission_Coalburn_?_CN_143384076_400000_CN_97551518_400000/LConn3 -- bus16/LConn1 -- _CN_143384076_400000_CN_284874050_400000/LConn3 -- _CN_143384076_400000_CN_100077745_400000/LConn3 -- _CN_143384076_400000_CN_308653841_400000/LConn3 -- _CN_143384076_400000_CN_86071326_400000/LConn3 -- _CN_143384076_400000_CN_91038272_400000/LConn3 -- _CN_143384076_400000_CN_143398452_400000/LConn3 -- _CN_143384076_400000_CN_308653843_400000/LConn3
  T_143383456_400000;132000_Coalburn_Substation/LConn1 -- _CN_143384076_400000_CN_143383456_400000/RConn1
  T_143383456_400000;132000_Coalburn_Substation/LConn2 -- _CN_143384076_400000_CN_143383456_400000/RConn2
  _CN_143384076_400000_CN_143383456_400000/RConn3 -- T_143383456_400000;132000_Coalburn_Substation/LConn3 -- bus17/LConn1
  _CN_143384076_400000_CN_284874050_400000/RConn1 -- T_284874050_400000_/LConn1 -- _CN_143219044_400000_CN_284874050_400000/LConn1
  _CN_143384076_400000_CN_284874050_400000/RConn2 -- T_284874050_400000_/LConn2 -- _CN_143219044_400000_CN_284874050_400000/LConn2
  _CN_143384076_400000_CN_284874050_400000/RConn3 -- T_284874050_400000_/LConn3 -- _CN_143219044_400000_CN_284874050_400000/LConn3 -- bus18/LConn1
  T_100077745_400000;275000_Kilmarnock_South_Substation/LConn1 -- _CN_143384076_400000_CN_100077745_400000/RConn1
  T_100077745_400000;275000_Kilmarnock_South_Substation/LConn2 -- _CN_143384076_400000_CN_100077745_400000/RConn2
  _CN_143384076_400000_CN_100077745_400000/RConn3 -- T_100077745_400000;275000_Kilmarnock_South_Substation/LConn3 -- bus19/LConn1
  _CN_143384076_400000_CN_308653841_400000/RConn1 -- T_308653841__/LConn1 -- _CN_308653840_400000_CN_308653841_400000/LConn1
  _CN_143384076_400000_CN_308653841_400000/RConn2 -- T_308653841__/LConn2 -- _CN_308653840_400000_CN_308653841_400000/LConn2
  _CN_143384076_400000_CN_308653841_400000/RConn3 -- T_308653841__/LConn3 -- _CN_308653840_400000_CN_308653841_400000/LConn3 -- bus20/LConn1
  T_86071326_400000;275000;132000_Windyhill_Substation/LConn1 -- _CN_143384076_400000_CN_86071326_400000/RConn1
  T_86071326_400000;275000;132000_Windyhill_Substation/LConn2 -- _CN_143384076_400000_CN_86071326_400000/RConn2
  _CN_143384076_400000_CN_86071326_400000/RConn3 -- T_86071326_400000;275000;132000_Windyhill_Substation/LConn3 -- bus21/LConn1
  T_91038272_400000_Inverkip_Substation/LConn1 -- _CN_143384076_400000_CN_91038272_400000/RConn1
  T_91038272_400000_Inverkip_Substation/LConn2 -- _CN_143384076_400000_CN_91038272_400000/RConn2
  _CN_143384076_400000_CN_91038272_400000/RConn3 -- T_91038272_400000_Inverkip_Substation/LConn3 -- bus22/LConn1
  T_143398452_400000_Neilston/LConn1 -- _CN_143384076_400000_CN_143398452_400000/RConn1
  T_143398452_400000_Neilston/LConn2 -- _CN_143384076_400000_CN_143398452_400000/RConn2
  _CN_143384076_400000_CN_143398452_400000/RConn3 -- T_143398452_400000_Neilston/LConn3 -- bus23/LConn1
  _CN_143384076_400000_CN_308653843_400000/RConn1 -- T_308653843_400000_/LConn1 -- _CN_304620087_400000_CN_308653843_400000/LConn1
  _CN_143384076_400000_CN_308653843_400000/RConn2 -- T_308653843_400000_/LConn2 -- _CN_304620087_400000_CN_308653843_400000/LConn2
  _CN_143384076_400000_CN_308653843_400000/RConn3 -- T_308653843_400000_/LConn3 -- _CN_304620087_400000_CN_308653843_400000/LConn3 -- bus24/LConn1
  T_96905262_400000;275000_/LConn1 -- SP_Transmission_Coalburn_?_CN_143384076_400000_CN_96905262_400000/RConn1
  T_96905262_400000;275000_/LConn2 -- SP_Transmission_Coalburn_?_CN_143384076_400000_CN_96905262_400000/RConn2
  SP_Transmission_Coalburn_?_CN_143384076_400000_CN_96905262_400000/RConn3 -- T_96905262_400000;275000_/LConn3 -- bus25/LConn1
  T_262532045_400000_/LConn1 -- SP_Transmission_Coalburn_?_CN_143384076_400000_CN_262532045_400000/RConn1
  T_262532045_400000_/LConn2 -- SP_Transmission_Coalburn_?_CN_143384076_400000_CN_262532045_400000/RConn2
  SP_Transmission_Coalburn_?_CN_143384076_400000_CN_262532045_400000/RConn3 -- T_262532045_400000_/LConn3 -- bus26/LConn1
  T_262523325_400000;132000_/LConn1 -- SP_Transmission_Coalburn_?_CN_143384076_400000_CN_262523325_400000/RConn1
  T_262523325_400000;132000_/LConn2 -- SP_Transmission_Coalburn_?_CN_143384076_400000_CN_262523325_400000/RConn2
  SP_Transmission_Coalburn_?_CN_143384076_400000_CN_262523325_400000/RConn3 -- T_262523325_400000;132000_/LConn3 -- bus27/LConn1
  SP_Transmission_Coalburn_?_CN_143384076_400000_CN_97551518_400000/RConn1 -- T_97551518__/LConn1 -- _CN_97551518_400000_CN_91104903_400000/LConn1
  SP_Transmission_Coalburn_?_CN_143384076_400000_CN_97551518_400000/RConn2 -- T_97551518__/LConn2 -- _CN_97551518_400000_CN_91104903_400000/LConn2
  SP_Transmission_Coalburn_?_CN_143384076_400000_CN_97551518_400000/RConn3 -- T_97551518__/LConn3 -- _CN_97551518_400000_CN_91104903_400000/LConn3 -- bus28/LConn1
  _CN_77065229_400000_CN_264650844_400000/LConn1 -- T_77065229_400000;132000_Stocking_Pelham_Substation/LConn1 -- _CN_77065229_400000_CN_24165071_400000/LConn1 -- _CN_77065229_400000_CN_25422135_400000/LConn1 -- _CN_77065229_400000_CN_29111908_400000/LConn1 -- _CN_77065229_400000_CN_29111844_400000/LConn1 -- _CN_77065229_400000_CN_25935453_400000/LConn1 -- _CN_77065229_400000_CN_38528291_400000/LConn1 -- _CN_77065229_400000_CN_25385285_400000/LConn1 -- _CN_77065229_400000_CN_22975329_400000/LConn1
  _CN_77065229_400000_CN_264650844_400000/LConn2 -- T_77065229_400000;132000_Stocking_Pelham_Substation/LConn2 -- _CN_77065229_400000_CN_24165071_400000/LConn2 -- _CN_77065229_400000_CN_25422135_400000/LConn2 -- _CN_77065229_400000_CN_29111908_400000/LConn2 -- _CN_77065229_400000_CN_29111844_400000/LConn2 -- _CN_77065229_400000_CN_25935453_400000/LConn2 -- _CN_77065229_400000_CN_38528291_400000/LConn2 -- _CN_77065229_400000_CN_25385285_400000/LConn2 -- _CN_77065229_400000_CN_22975329_400000/LConn2
  _CN_77065229_400000_CN_264650844_400000/LConn3 -- T_77065229_400000;132000_Stocking_Pelham_Substation/LConn3 -- _CN_77065229_400000_CN_24165071_400000/LConn3 -- bus29/LConn1 -- _CN_77065229_400000_CN_25422135_400000/LConn3 -- _CN_77065229_400000_CN_29111908_400000/LConn3 -- _CN_77065229_400000_CN_29111844_400000/LConn3 -- _CN_77065229_400000_CN_25935453_400000/LConn3 -- _CN_77065229_400000_CN_38528291_400000/LConn3 -- _CN_77065229_400000_CN_25385285_400000/LConn3 -- _CN_77065229_400000_CN_22975329_400000/LConn3
  _CN_77065229_400000_CN_264650844_400000/RConn1 -- T_264650844_400000_/LConn1 -- _CN_264650844_400000_CN_264650878_400000/LConn1 -- _CN_264650844_400000_CN_25422135_400000/LConn1
  _CN_77065229_400000_CN_264650844_400000/RConn2 -- T_264650844_400000_/LConn2 -- _CN_264650844_400000_CN_264650878_400000/LConn2 -- _CN_264650844_400000_CN_25422135_400000/LConn2
  _CN_77065229_400000_CN_264650844_400000/RConn3 -- T_264650844_400000_/LConn3 -- _CN_264650844_400000_CN_264650878_400000/LConn3 -- _CN_264650844_400000_CN_25422135_400000/LConn3 -- bus30/LConn1
  _CN_77065229_400000_CN_25422135_400000/RConn1 -- T_25422135_400000;132000_Bramford_Substation/LConn1 -- _CN_264650844_400000_CN_25422135_400000/RConn1
  _CN_77065229_400000_CN_25422135_400000/RConn2 -- T_25422135_400000;132000_Bramford_Substation/LConn2 -- _CN_264650844_400000_CN_25422135_400000/RConn2
  _CN_77065229_400000_CN_25422135_400000/RConn3 -- T_25422135_400000;132000_Bramford_Substation/LConn3 -- _CN_264650844_400000_CN_25422135_400000/RConn3 -- bus31/LConn1
  T_29111908_400000;132000_Braintree_Substation/LConn1 -- _CN_77065229_400000_CN_29111908_400000/RConn1
  T_29111908_400000;132000_Braintree_Substation/LConn2 -- _CN_77065229_400000_CN_29111908_400000/RConn2
  _CN_77065229_400000_CN_29111908_400000/RConn3 -- T_29111908_400000;132000_Braintree_Substation/LConn3 -- bus32/LConn1
  _CN_77065229_400000_CN_29111844_400000/RConn1 -- T_29111844_400000;132000_Rayleigh_Main_Substation/LConn1 -- National_Grid_CN_29111844_400000_CN_100773252_400000/LConn1 -- National_Grid_CN_29111844_400000_CN_94530230_400000/LConn1 -- National_Grid_CN_29111844_400000_CN_264214748_400000/LConn1
  _CN_77065229_400000_CN_29111844_400000/RConn2 -- T_29111844_400000;132000_Rayleigh_Main_Substation/LConn2 -- National_Grid_CN_29111844_400000_CN_100773252_400000/LConn2 -- National_Grid_CN_29111844_400000_CN_94530230_400000/LConn2 -- National_Grid_CN_29111844_400000_CN_264214748_400000/LConn2
  _CN_77065229_400000_CN_29111844_400000/RConn3 -- T_29111844_400000;132000_Rayleigh_Main_Substation/LConn3 -- National_Grid_CN_29111844_400000_CN_100773252_400000/LConn3 -- National_Grid_CN_29111844_400000_CN_94530230_400000/LConn3 -- National_Grid_CN_29111844_400000_CN_264214748_400000/LConn3 -- bus33/LConn1
  T_25935453_400000;132000_Burwell_Main_Substation_(BURW)/LConn1 -- _CN_77065229_400000_CN_25935453_400000/RConn1
  T_25935453_400000;132000_Burwell_Main_Substation_(BURW)/LConn2 -- _CN_77065229_400000_CN_25935453_400000/RConn2
  _CN_77065229_400000_CN_25935453_400000/RConn3 -- T_25935453_400000;132000_Burwell_Main_Substation_(BURW)/LConn3 -- bus34/LConn1
  _CN_77065229_400000_CN_38528291_400000/RConn1 -- T_38528291_400000;132000_Walpole_Substation/LConn1 -- _CN_38528291_400000_CN_32227788_400000/LConn1 -- _CN_38528291_400000_CN_143902275_400000/RConn1 -- _CN_38528291_400000_CN_190511290_400000/LConn1
  _CN_77065229_400000_CN_38528291_400000/RConn2 -- T_38528291_400000;132000_Walpole_Substation/LConn2 -- _CN_38528291_400000_CN_32227788_400000/LConn2 -- _CN_38528291_400000_CN_143902275_400000/RConn2 -- _CN_38528291_400000_CN_190511290_400000/LConn2
  _CN_77065229_400000_CN_38528291_400000/RConn3 -- T_38528291_400000;132000_Walpole_Substation/LConn3 -- _CN_38528291_400000_CN_32227788_400000/LConn3 -- bus35/LConn1 -- _CN_38528291_400000_CN_143902275_400000/RConn3 -- _CN_38528291_400000_CN_190511290_400000/LConn3
  T_25385285__Rye_House_Substation/LConn1 -- _CN_77065229_400000_CN_25385285_400000/RConn1
  T_25385285__Rye_House_Substation/LConn2 -- _CN_77065229_400000_CN_25385285_400000/RConn2
  _CN_77065229_400000_CN_25385285_400000/RConn3 -- T_25385285__Rye_House_Substation/LConn3 -- bus36/LConn1
  T_22975329_400000;275000_Waltham_Cross_Substation/LConn1 -- _CN_77065229_400000_CN_22975329_400000/RConn1
  T_22975329_400000;275000_Waltham_Cross_Substation/LConn2 -- _CN_77065229_400000_CN_22975329_400000/RConn2
  _CN_77065229_400000_CN_22975329_400000/RConn3 -- T_22975329_400000;275000_Waltham_Cross_Substation/LConn3 -- bus37/LConn1
  _CN_77065229_400000_CN_24165071_400000/RConn1 -- T_24165071_400000_Wymondley_Substation/LConn1 -- _CN_41809491_400000_CN_24165071_400000/LConn1 -- _CN_24165071_400000_CN_89038614_400000/LConn1 -- _CN_24165071_400000_CN_154635235_400000/LConn1
  _CN_77065229_400000_CN_24165071_400000/RConn2 -- T_24165071_400000_Wymondley_Substation/LConn2 -- _CN_41809491_400000_CN_24165071_400000/LConn2 -- _CN_24165071_400000_CN_89038614_400000/LConn2 -- _CN_24165071_400000_CN_154635235_400000/LConn2
  _CN_77065229_400000_CN_24165071_400000/RConn3 -- T_24165071_400000_Wymondley_Substation/LConn3 -- _CN_41809491_400000_CN_24165071_400000/LConn3 -- _CN_24165071_400000_CN_89038614_400000/LConn3 -- _CN_24165071_400000_CN_154635235_400000/LConn3 -- bus38/LConn1
  _CN_97256377_400000_CN_81048391_400000/LConn1 -- T_97256377_400000;275000_/LConn1 -- _CN_97256377_400000_CN_55578199_400000/LConn1 -- _CN_97256377_400000_CN_92529432_400000/LConn1 -- _CN_97256377_400000_CN_92676046_400000/LConn1 -- _CN_97256377_400000_CN_92737152_400000/LConn1 -- _CN_97256377_400000_CN_293584682_400000/LConn1
  _CN_97256377_400000_CN_81048391_400000/LConn2 -- T_97256377_400000;275000_/LConn2 -- _CN_97256377_400000_CN_55578199_400000/LConn2 -- _CN_97256377_400000_CN_92529432_400000/LConn2 -- _CN_97256377_400000_CN_92676046_400000/LConn2 -- _CN_97256377_400000_CN_92737152_400000/LConn2 -- _CN_97256377_400000_CN_293584682_400000/LConn2
  _CN_97256377_400000_CN_81048391_400000/LConn3 -- T_97256377_400000;275000_/LConn3 -- _CN_97256377_400000_CN_55578199_400000/LConn3 -- _CN_97256377_400000_CN_92529432_400000/LConn3 -- _CN_97256377_400000_CN_92676046_400000/LConn3 -- _CN_97256377_400000_CN_92737152_400000/LConn3 -- _CN_97256377_400000_CN_293584682_400000/LConn3 -- bus39/LConn1
  _CN_97256377_400000_CN_81048391_400000/RConn1 -- T_81048391_400000;275000;132000_Penwortham_Substation/LConn1 -- National_Grid_Penwortham_Stanah_CN_310495264_400000_CN_81048391_400000/LConn1 -- _CN_45357172_400000_CN_81048391_400000/LConn1
  _CN_97256377_400000_CN_81048391_400000/RConn2 -- T_81048391_400000;275000;132000_Penwortham_Substation/LConn2 -- National_Grid_Penwortham_Stanah_CN_310495264_400000_CN_81048391_400000/LConn2 -- _CN_45357172_400000_CN_81048391_400000/LConn2
  _CN_97256377_400000_CN_81048391_400000/RConn3 -- T_81048391_400000;275000;132000_Penwortham_Substation/LConn3 -- National_Grid_Penwortham_Stanah_CN_310495264_400000_CN_81048391_400000/LConn3 -- _CN_45357172_400000_CN_81048391_400000/LConn3 -- bus40/LConn1
  _CN_97256377_400000_CN_55578199_400000/RConn1 -- T_55578199_400000_Padiham_Substation/LConn1 -- _CN_55578199_400000_CN_142841192_400000/LConn1 -- _CN_55578199_400000_CN_90547674_400000/LConn1
  _CN_97256377_400000_CN_55578199_400000/RConn2 -- T_55578199_400000_Padiham_Substation/LConn2 -- _CN_55578199_400000_CN_142841192_400000/LConn2 -- _CN_55578199_400000_CN_90547674_400000/LConn2
  _CN_97256377_400000_CN_55578199_400000/RConn3 -- T_55578199_400000_Padiham_Substation/LConn3 -- _CN_55578199_400000_CN_142841192_400000/LConn3 -- _CN_55578199_400000_CN_90547674_400000/LConn3 -- bus41/LConn1
  _CN_97256377_400000_CN_92529432_400000/RConn1 -- T_92529432_400000_Daines_Substation/LConn1 -- National_Grid_Daines_Macclesfield_CN_142738881_400000_CN_92529432_400000/LConn1 -- _CN_92529432_400000_CN_365868376_400000/LConn1 -- _CN_92529432_400000_CN_293584682_400000/LConn1 -- _CN_92529432_400000_CN_92676046_400000/LConn1
  _CN_97256377_400000_CN_92529432_400000/RConn2 -- T_92529432_400000_Daines_Substation/LConn2 -- National_Grid_Daines_Macclesfield_CN_142738881_400000_CN_92529432_400000/LConn2 -- _CN_92529432_400000_CN_365868376_400000/LConn2 -- _CN_92529432_400000_CN_293584682_400000/LConn2 -- _CN_92529432_400000_CN_92676046_400000/LConn2
  _CN_97256377_400000_CN_92529432_400000/RConn3 -- T_92529432_400000_Daines_Substation/LConn3 -- National_Grid_Daines_Macclesfield_CN_142738881_400000_CN_92529432_400000/LConn3 -- _CN_92529432_400000_CN_365868376_400000/LConn3 -- _CN_92529432_400000_CN_293584682_400000/LConn3 -- _CN_92529432_400000_CN_92676046_400000/LConn3 -- bus42/LConn1
  _CN_97256377_400000_CN_92676046_400000/RConn1 -- T_92676046_400000;132000_/LConn1 -- _CN_92529432_400000_CN_92676046_400000/RConn1
  _CN_97256377_400000_CN_92676046_400000/RConn2 -- T_92676046_400000;132000_/LConn2 -- _CN_92529432_400000_CN_92676046_400000/RConn2
  _CN_97256377_400000_CN_92676046_400000/RConn3 -- T_92676046_400000;132000_/LConn3 -- _CN_92529432_400000_CN_92676046_400000/RConn3 -- bus43/LConn1
  _CN_97256377_400000_CN_92737152_400000/RConn1 -- T_92737152_400000_/LConn1 -- _CN_92737152_400000_CN_293585872_400000/LConn1
  _CN_97256377_400000_CN_92737152_400000/RConn2 -- T_92737152_400000_/LConn2 -- _CN_92737152_400000_CN_293585872_400000/LConn2
  _CN_97256377_400000_CN_92737152_400000/RConn3 -- T_92737152_400000_/LConn3 -- _CN_92737152_400000_CN_293585872_400000/LConn3 -- bus44/LConn1
  _CN_97256377_400000_CN_293584682_400000/RConn1 -- T_293584682__/LConn1 -- _CN_92529432_400000_CN_293584682_400000/RConn1
  _CN_97256377_400000_CN_293584682_400000/RConn2 -- T_293584682__/LConn2 -- _CN_92529432_400000_CN_293584682_400000/RConn2
  _CN_97256377_400000_CN_293584682_400000/RConn3 -- T_293584682__/LConn3 -- _CN_92529432_400000_CN_293584682_400000/RConn3 -- bus45/LConn1
  Woodhead_Tunnel_3_CN_159038999_400000_CN_291629706_400000/LConn1 -- T_159038999_400000_/LConn1 -- _CN_159038999_400000_CN_90539508_400000/LConn1 -- _CN_159038999_400000_CN_101077623_400000/LConn1 -- _CN_159038999_400000_CN_313495303_400000/LConn1 -- _CN_159038999_400000_CN_34383059_400000/LConn1 -- _CN_159038999_400000_CN_90547679_400000/LConn1
  Woodhead_Tunnel_3_CN_159038999_400000_CN_291629706_400000/LConn2 -- T_159038999_400000_/LConn2 -- _CN_159038999_400000_CN_90539508_400000/LConn2 -- _CN_159038999_400000_CN_101077623_400000/LConn2 -- _CN_159038999_400000_CN_313495303_400000/LConn2 -- _CN_159038999_400000_CN_34383059_400000/LConn2 -- _CN_159038999_400000_CN_90547679_400000/LConn2
  Woodhead_Tunnel_3_CN_159038999_400000_CN_291629706_400000/LConn3 -- T_159038999_400000_/LConn3 -- _CN_159038999_400000_CN_90539508_400000/LConn3 -- _CN_159038999_400000_CN_101077623_400000/LConn3 -- _CN_159038999_400000_CN_313495303_400000/LConn3 -- _CN_159038999_400000_CN_34383059_400000/LConn3 -- _CN_159038999_400000_CN_90547679_400000/LConn3 -- bus46/LConn1
  Woodhead_Tunnel_3_CN_159038999_400000_CN_291629706_400000/RConn1 -- T_291629706__/LConn1 -- _CN_291629706_400000_CN_147672722_400000/LConn1
  Woodhead_Tunnel_3_CN_159038999_400000_CN_291629706_400000/RConn2 -- T_291629706__/LConn2 -- _CN_291629706_400000_CN_147672722_400000/LConn2
  Woodhead_Tunnel_3_CN_159038999_400000_CN_291629706_400000/RConn3 -- T_291629706__/LConn3 -- _CN_291629706_400000_CN_147672722_400000/LConn3 -- bus47/LConn1
  T_90539508_400000_/LConn1 -- _CN_159038999_400000_CN_90539508_400000/RConn1
  T_90539508_400000_/LConn2 -- _CN_159038999_400000_CN_90539508_400000/RConn2
  _CN_159038999_400000_CN_90539508_400000/RConn3 -- T_90539508_400000_/LConn3 -- bus48/LConn1
  T_101077623_400000;275000_/LConn1 -- _CN_159038999_400000_CN_101077623_400000/RConn1
  T_101077623_400000;275000_/LConn2 -- _CN_159038999_400000_CN_101077623_400000/RConn2
  _CN_159038999_400000_CN_101077623_400000/RConn3 -- T_101077623_400000;275000_/LConn3 -- bus49/LConn1
  T_313495303__/LConn1 -- _CN_159038999_400000_CN_313495303_400000/RConn1
  T_313495303__/LConn2 -- _CN_159038999_400000_CN_313495303_400000/RConn2
  _CN_159038999_400000_CN_313495303_400000/RConn3 -- T_313495303__/LConn3 -- bus50/LConn1
  _CN_159038999_400000_CN_34383059_400000/RConn1 -- G_34383059_Eggborough_Power_Station/RConn1 -- _CN_313495269_400000_CN_34383059_400000/LConn1
  _CN_159038999_400000_CN_34383059_400000/RConn2 -- G_34383059_Eggborough_Power_Station/RConn2 -- _CN_313495269_400000_CN_34383059_400000/LConn2
  _CN_159038999_400000_CN_34383059_400000/RConn3 -- G_34383059_Eggborough_Power_Station/RConn3 -- _CN_313495269_400000_CN_34383059_400000/LConn3 -- bus51/LConn1
  _CN_159038999_400000_CN_90547679_400000/RConn1 -- T_90547679_400000_/LConn1 -- _CN_100861711_400000_CN_90547679_400000/LConn1
  _CN_159038999_400000_CN_90547679_400000/RConn2 -- T_90547679_400000_/LConn2 -- _CN_100861711_400000_CN_90547679_400000/LConn2
  _CN_159038999_400000_CN_90547679_400000/RConn3 -- T_90547679_400000_/LConn3 -- _CN_100861711_400000_CN_90547679_400000/LConn3 -- bus52/LConn1
  _CN_102198808_400000_CN_308788887_400000/LConn1 -- T_102198808_400000;132000_Eccles_Substation/LConn1 -- _CN_102198808_400000_CN_310502642_400000/LConn1 -- _CN_102198808_400000_CN_91955171_400000/LConn1 -- _CN_102198808_400000_CN_97551523_400000/LConn1
  _CN_102198808_400000_CN_308788887_400000/LConn2 -- T_102198808_400000;132000_Eccles_Substation/LConn2 -- _CN_102198808_400000_CN_310502642_400000/LConn2 -- _CN_102198808_400000_CN_91955171_400000/LConn2 -- _CN_102198808_400000_CN_97551523_400000/LConn2
  _CN_102198808_400000_CN_308788887_400000/LConn3 -- T_102198808_400000;132000_Eccles_Substation/LConn3 -- _CN_102198808_400000_CN_310502642_400000/LConn3 -- _CN_102198808_400000_CN_91955171_400000/LConn3 -- _CN_102198808_400000_CN_97551523_400000/LConn3 -- bus53/LConn1
  T_308788887_400000_/LConn1 -- _CN_102198808_400000_CN_308788887_400000/RConn1
  T_308788887_400000_/LConn2 -- _CN_102198808_400000_CN_308788887_400000/RConn2
  _CN_102198808_400000_CN_308788887_400000/RConn3 -- T_308788887_400000_/LConn3 -- bus54/LConn1
  T_310502642_400000;275000_/LConn1 -- _CN_102198808_400000_CN_310502642_400000/RConn1
  T_310502642_400000;275000_/LConn2 -- _CN_102198808_400000_CN_310502642_400000/RConn2
  _CN_102198808_400000_CN_310502642_400000/RConn3 -- T_310502642_400000;275000_/LConn3 -- bus55/LConn1
  _CN_102198808_400000_CN_91955171_400000/RConn1 -- T_91955171_400000;275000;132000_Stella_West_Sub_Station/LConn1 -- _CN_220798107_400000_CN_91955171_400000/LConn1
  _CN_102198808_400000_CN_91955171_400000/RConn2 -- T_91955171_400000;275000;132000_Stella_West_Sub_Station/LConn2 -- _CN_220798107_400000_CN_91955171_400000/LConn2
  _CN_102198808_400000_CN_91955171_400000/RConn3 -- T_91955171_400000;275000;132000_Stella_West_Sub_Station/LConn3 -- _CN_220798107_400000_CN_91955171_400000/LConn3 -- bus56/LConn1
  _CN_102198808_400000_CN_97551523_400000/RConn1 -- T_97551523__/LConn1 -- _CN_97551523_400000_CN_91104903_400000/LConn1
  _CN_102198808_400000_CN_97551523_400000/RConn2 -- T_97551523__/LConn2 -- _CN_97551523_400000_CN_91104903_400000/LConn2
  _CN_102198808_400000_CN_97551523_400000/RConn3 -- T_97551523__/LConn3 -- _CN_97551523_400000_CN_91104903_400000/LConn3 -- bus57/LConn1
  _CN_314338845_400000_CN_143905069_400000/LConn1 -- T_314338845__/LConn1 -- _CN_314338845_400000_CN_91003253_400000/LConn1 -- _CN_314338845_400000_CN_35287066_400000/LConn1 -- _CN_314338845_400000_CN_314338790_400000/LConn1 -- _CN_314338845_400000_CN_314338851_400000/LConn1 -- _CN_314338845_400000_CN_314338849_400000/LConn1
  _CN_314338845_400000_CN_143905069_400000/LConn2 -- T_314338845__/LConn2 -- _CN_314338845_400000_CN_91003253_400000/LConn2 -- _CN_314338845_400000_CN_35287066_400000/LConn2 -- _CN_314338845_400000_CN_314338790_400000/LConn2 -- _CN_314338845_400000_CN_314338851_400000/LConn2 -- _CN_314338845_400000_CN_314338849_400000/LConn2
  _CN_314338845_400000_CN_143905069_400000/LConn3 -- T_314338845__/LConn3 -- _CN_314338845_400000_CN_91003253_400000/LConn3 -- _CN_314338845_400000_CN_35287066_400000/LConn3 -- _CN_314338845_400000_CN_314338790_400000/LConn3 -- _CN_314338845_400000_CN_314338851_400000/LConn3 -- _CN_314338845_400000_CN_314338849_400000/LConn3 -- bus58/LConn1
  T_143905069_400000;275000_High_Marnham_Substation/LConn1 -- _CN_314338845_400000_CN_143905069_400000/RConn1
  T_143905069_400000;275000_High_Marnham_Substation/LConn2 -- _CN_314338845_400000_CN_143905069_400000/RConn2
  _CN_314338845_400000_CN_143905069_400000/RConn3 -- T_143905069_400000;275000_High_Marnham_Substation/LConn3 -- bus59/LConn1
  _CN_314338845_400000_CN_91003253_400000/RConn1 -- T_91003253_400000;132000_Staythorpe_Substation/LConn1 -- _CN_314338790_400000_CN_91003253_400000/LConn1 -- _CN_91003253_400000_CN_88287125_400000/LConn1
  _CN_314338845_400000_CN_91003253_400000/RConn2 -- T_91003253_400000;132000_Staythorpe_Substation/LConn2 -- _CN_314338790_400000_CN_91003253_400000/LConn2 -- _CN_91003253_400000_CN_88287125_400000/LConn2
  _CN_314338845_400000_CN_91003253_400000/RConn3 -- T_91003253_400000;132000_Staythorpe_Substation/LConn3 -- _CN_314338790_400000_CN_91003253_400000/LConn3 -- _CN_91003253_400000_CN_88287125_400000/LConn3 -- bus60/LConn1
  _CN_314338845_400000_CN_35287066_400000/RConn1 -- G_35287066_Ratcliffe_Power_Station/RConn1 -- _CN_87204522_400000_CN_35287066_400000/LConn1 -- _CN_71118628_400000_CN_35287066_400000/LConn1 -- _CN_90534270_400000_CN_35287066_400000/LConn1 -- _CN_315965849_400000_CN_35287066_400000/LConn1 -- _CN_277887478_400000_CN_35287066_400000/LConn1
  _CN_314338845_400000_CN_35287066_400000/RConn2 -- G_35287066_Ratcliffe_Power_Station/RConn2 -- _CN_87204522_400000_CN_35287066_400000/LConn2 -- _CN_71118628_400000_CN_35287066_400000/LConn2 -- _CN_90534270_400000_CN_35287066_400000/LConn2 -- _CN_315965849_400000_CN_35287066_400000/LConn2 -- _CN_277887478_400000_CN_35287066_400000/LConn2
  _CN_314338845_400000_CN_35287066_400000/RConn3 -- G_35287066_Ratcliffe_Power_Station/RConn3 -- _CN_87204522_400000_CN_35287066_400000/LConn3 -- _CN_71118628_400000_CN_35287066_400000/LConn3 -- _CN_90534270_400000_CN_35287066_400000/LConn3 -- _CN_315965849_400000_CN_35287066_400000/LConn3 -- _CN_277887478_400000_CN_35287066_400000/LConn3 -- bus61/LConn1
  _CN_314338845_400000_CN_314338790_400000/RConn1 -- T_314338790_400000_/LConn1 -- _CN_314338849_400000_CN_314338790_400000/LConn1 -- _CN_314338790_400000_CN_91003253_400000/RConn1 -- _CN_314338790_400000_CN_402566315_400000/LConn1
  _CN_314338845_400000_CN_314338790_400000/RConn2 -- T_314338790_400000_/LConn2 -- _CN_314338849_400000_CN_314338790_400000/LConn2 -- _CN_314338790_400000_CN_91003253_400000/RConn2 -- _CN_314338790_400000_CN_402566315_400000/LConn2
  _CN_314338845_400000_CN_314338790_400000/RConn3 -- T_314338790_400000_/LConn3 -- _CN_314338849_400000_CN_314338790_400000/LConn3 -- _CN_314338790_400000_CN_91003253_400000/RConn3 -- _CN_314338790_400000_CN_402566315_400000/LConn3 -- bus62/LConn1
  T_314338851__/LConn1 -- _CN_314338845_400000_CN_314338851_400000/RConn1
  T_314338851__/LConn2 -- _CN_314338845_400000_CN_314338851_400000/RConn2
  _CN_314338845_400000_CN_314338851_400000/RConn3 -- T_314338851__/LConn3 -- bus63/LConn1
  _CN_314338845_400000_CN_314338849_400000/RConn1 -- T_314338849__/LConn1 -- _CN_314338849_400000_CN_314338790_400000/RConn1
  _CN_314338845_400000_CN_314338849_400000/RConn2 -- T_314338849__/LConn2 -- _CN_314338849_400000_CN_314338790_400000/RConn2
  _CN_314338845_400000_CN_314338849_400000/RConn3 -- T_314338849__/LConn3 -- _CN_314338849_400000_CN_314338790_400000/RConn3 -- bus64/LConn1
  National_Grid_Penwortham_Stanah_CN_310495264_400000_CN_81048391_400000/RConn1 -- T_310495264_400000;132000_Stanah_Substation/LConn1 -- National_Grid_Penwortham_Stanah_CN_310495264_400000_CN_94004582_400000/LConn1
  National_Grid_Penwortham_Stanah_CN_310495264_400000_CN_81048391_400000/RConn2 -- T_310495264_400000;132000_Stanah_Substation/LConn2 -- National_Grid_Penwortham_Stanah_CN_310495264_400000_CN_94004582_400000/LConn2
  National_Grid_Penwortham_Stanah_CN_310495264_400000_CN_81048391_400000/RConn3 -- T_310495264_400000;132000_Stanah_Substation/LConn3 -- National_Grid_Penwortham_Stanah_CN_310495264_400000_CN_94004582_400000/LConn3 -- bus65/LConn1
  National_Grid_Penwortham_Stanah_CN_310495264_400000_CN_94004582_400000/RConn1 -- T_94004582_400000_Heysham_Substation/LConn1 -- _CN_94004582_400000_CN_310488541_400000/LConn1 -- _CN_94004582_400000_CN_310488542_400000/LConn1 -- _CN_45357172_400000_CN_94004582_400000/LConn1
  National_Grid_Penwortham_Stanah_CN_310495264_400000_CN_94004582_400000/RConn2 -- T_94004582_400000_Heysham_Substation/LConn2 -- _CN_94004582_400000_CN_310488541_400000/LConn2 -- _CN_94004582_400000_CN_310488542_400000/LConn2 -- _CN_45357172_400000_CN_94004582_400000/LConn2
  National_Grid_Penwortham_Stanah_CN_310495264_400000_CN_94004582_400000/RConn3 -- T_94004582_400000_Heysham_Substation/LConn3 -- _CN_94004582_400000_CN_310488541_400000/LConn3 -- _CN_94004582_400000_CN_310488542_400000/LConn3 -- bus66/LConn1 -- _CN_45357172_400000_CN_94004582_400000/LConn3
  T_100773252_400000_/LConn1 -- National_Grid_CN_29111844_400000_CN_100773252_400000/RConn1
  T_100773252_400000_/LConn2 -- National_Grid_CN_29111844_400000_CN_100773252_400000/RConn2
  National_Grid_CN_29111844_400000_CN_100773252_400000/RConn3 -- T_100773252_400000_/LConn3 -- bus67/LConn1
  T_94530230_400000;275000_Tilbury_Substation/LConn1 -- National_Grid_CN_29111844_400000_CN_94530230_400000/RConn1
  T_94530230_400000;275000_Tilbury_Substation/LConn2 -- National_Grid_CN_29111844_400000_CN_94530230_400000/RConn2
  National_Grid_CN_29111844_400000_CN_94530230_400000/RConn3 -- T_94530230_400000;275000_Tilbury_Substation/LConn3 -- bus68/LConn1
  National_Grid_CN_29111844_400000_CN_264214748_400000/RConn1 -- T_264214748__/LConn1 -- _CN_264214748_400000_CN_103829261_400000/LConn1
  National_Grid_CN_29111844_400000_CN_264214748_400000/RConn2 -- T_264214748__/LConn2 -- _CN_264214748_400000_CN_103829261_400000/LConn2
  National_Grid_CN_29111844_400000_CN_264214748_400000/RConn3 -- T_264214748__/LConn3 -- _CN_264214748_400000_CN_103829261_400000/LConn3 -- bus69/LConn1
  _CN_164380199_400000_CN_193460871_400000/LConn1 -- T_164380199_400000;132000_Elland_Substation/LConn1 -- _CN_164380199_400000_CN_163036722_400000/LConn1 -- _CN_164380199_400000_CN_193617444_400000/LConn1
  _CN_164380199_400000_CN_193460871_400000/LConn2 -- T_164380199_400000;132000_Elland_Substation/LConn2 -- _CN_164380199_400000_CN_163036722_400000/LConn2 -- _CN_164380199_400000_CN_193617444_400000/LConn2
  _CN_164380199_400000_CN_193460871_400000/LConn3 -- T_164380199_400000;132000_Elland_Substation/LConn3 -- _CN_164380199_400000_CN_163036722_400000/LConn3 -- bus70/LConn1 -- _CN_164380199_400000_CN_193617444_400000/LConn3
  T_193460871__/LConn1 -- _CN_164380199_400000_CN_193460871_400000/RConn1
  T_193460871__/LConn2 -- _CN_164380199_400000_CN_193460871_400000/RConn2
  _CN_164380199_400000_CN_193460871_400000/RConn3 -- T_193460871__/LConn3 -- bus71/LConn1
  _CN_164380199_400000_CN_193617444_400000/RConn1 -- T_193617444_400000_Ferrybridge_C_275kV_Substation/LConn1 -- _CN_193617444_400000_CN_313495307_400000/LConn1
  _CN_164380199_400000_CN_193617444_400000/RConn2 -- T_193617444_400000_Ferrybridge_C_275kV_Substation/LConn2 -- _CN_193617444_400000_CN_313495307_400000/LConn2
  _CN_164380199_400000_CN_193617444_400000/RConn3 -- T_193617444_400000_Ferrybridge_C_275kV_Substation/LConn3 -- _CN_193617444_400000_CN_313495307_400000/LConn3 -- bus72/LConn1
  T_163036722_400000_/LConn1 -- _CN_164380199_400000_CN_163036722_400000/RConn1
  T_163036722_400000_/LConn2 -- _CN_164380199_400000_CN_163036722_400000/RConn2
  _CN_164380199_400000_CN_163036722_400000/RConn3 -- T_163036722_400000_/LConn3 -- bus73/LConn1
  T_292220969_400000_/LConn1 -- _CN_292220969_400000_CN_143791249_400000/LConn1
  T_292220969_400000_/LConn2 -- _CN_292220969_400000_CN_143791249_400000/LConn2
  _CN_292220969_400000_CN_143791249_400000/LConn3 -- T_292220969_400000_/LConn3 -- bus74/LConn1
  _CN_292220969_400000_CN_143791249_400000/RConn1 -- T_143791249_400000;132000_Indian_Queens_Substation/LConn1 -- _CN_143791249_400000_CN_119616836_400000/LConn1 -- _CN_143791249_400000_CN_34656007_400000/LConn1 -- _CN_143791249_400000_CN_143791247_400000/LConn1 -- _CN_143791249_400000_CN_100009331_400000/LConn1
  _CN_292220969_400000_CN_143791249_400000/RConn2 -- T_143791249_400000;132000_Indian_Queens_Substation/LConn2 -- _CN_143791249_400000_CN_119616836_400000/LConn2 -- _CN_143791249_400000_CN_34656007_400000/LConn2 -- _CN_143791249_400000_CN_143791247_400000/LConn2 -- _CN_143791249_400000_CN_100009331_400000/LConn2
  _CN_292220969_400000_CN_143791249_400000/RConn3 -- T_143791249_400000;132000_Indian_Queens_Substation/LConn3 -- _CN_143791249_400000_CN_119616836_400000/LConn3 -- _CN_143791249_400000_CN_34656007_400000/LConn3 -- _CN_143791249_400000_CN_143791247_400000/LConn3 -- bus75/LConn1 -- _CN_143791249_400000_CN_100009331_400000/LConn3
  National_Grid_Grain_Kemsley_CN_109189895_400000_CN_109189893_400000/LConn1 -- T_109189895__/LConn1 -- National_Grid_Grain_Kemsley_CN_109189895_400000_CN_10270618_400000/LConn1
  National_Grid_Grain_Kemsley_CN_109189895_400000_CN_109189893_400000/LConn2 -- T_109189895__/LConn2 -- National_Grid_Grain_Kemsley_CN_109189895_400000_CN_10270618_400000/LConn2
  National_Grid_Grain_Kemsley_CN_109189895_400000_CN_109189893_400000/LConn3 -- T_109189895__/LConn3 -- National_Grid_Grain_Kemsley_CN_109189895_400000_CN_10270618_400000/LConn3 -- bus76/LConn1
  National_Grid_Grain_Kemsley_CN_109189895_400000_CN_109189893_400000/RConn1 -- T_109189893__/LConn1 -- National_Grid_Grain_Kemsley_CN_109189893_400000_CN_91010022_400000/LConn1
  National_Grid_Grain_Kemsley_CN_109189895_400000_CN_109189893_400000/RConn2 -- T_109189893__/LConn2 -- National_Grid_Grain_Kemsley_CN_109189893_400000_CN_91010022_400000/LConn2
  National_Grid_Grain_Kemsley_CN_109189895_400000_CN_109189893_400000/RConn3 -- T_109189893__/LConn3 -- National_Grid_Grain_Kemsley_CN_109189893_400000_CN_91010022_400000/LConn3 -- bus77/LConn1
  National_Grid_Grain_Kemsley_CN_109189895_400000_CN_10270618_400000/RConn1 -- G_10270618_/RConn1 -- _CN_143783006_400000_CN_10270618_400000/LConn1 -- National_Grid_Kingsnorth_Tilbury_CN_103829261_400000_CN_10270618_400000/LConn1
  National_Grid_Grain_Kemsley_CN_109189895_400000_CN_10270618_400000/RConn2 -- G_10270618_/RConn2 -- _CN_143783006_400000_CN_10270618_400000/LConn2 -- National_Grid_Kingsnorth_Tilbury_CN_103829261_400000_CN_10270618_400000/LConn2
  National_Grid_Grain_Kemsley_CN_109189895_400000_CN_10270618_400000/RConn3 -- G_10270618_/RConn3 -- _CN_143783006_400000_CN_10270618_400000/LConn3 -- National_Grid_Kingsnorth_Tilbury_CN_103829261_400000_CN_10270618_400000/LConn3 -- bus78/LConn1
  Nursling_Mannington_CN_23988786_400000_CN_20851038_400000/LConn1 -- T_23988786_400000_Nursling_Substation/LConn1 -- Nursling_Mannington_CN_23988786_400000_CN_90099036_400000/LConn1 -- Nursling_Mannington_CN_23988786_400000_CN_5728891_400000/LConn1
  Nursling_Mannington_CN_23988786_400000_CN_20851038_400000/LConn2 -- T_23988786_400000_Nursling_Substation/LConn2 -- Nursling_Mannington_CN_23988786_400000_CN_90099036_400000/LConn2 -- Nursling_Mannington_CN_23988786_400000_CN_5728891_400000/LConn2
  Nursling_Mannington_CN_23988786_400000_CN_20851038_400000/LConn3 -- T_23988786_400000_Nursling_Substation/LConn3 -- Nursling_Mannington_CN_23988786_400000_CN_90099036_400000/LConn3 -- bus79/LConn1 -- Nursling_Mannington_CN_23988786_400000_CN_5728891_400000/LConn3
  Nursling_Mannington_CN_23988786_400000_CN_20851038_400000/RConn1 -- T_20851038_400000;132000_Lovedean_Substation/LConn1 -- _CN_23300984_400000_CN_20851038_400000/LConn1 -- Bolney_Lovedean_CN_91082448_400000_CN_20851038_400000/LConn1 -- _CN_88389243_400000_CN_20851038_400000/LConn1
  Nursling_Mannington_CN_23988786_400000_CN_20851038_400000/RConn2 -- T_20851038_400000;132000_Lovedean_Substation/LConn2 -- _CN_23300984_400000_CN_20851038_400000/LConn2 -- Bolney_Lovedean_CN_91082448_400000_CN_20851038_400000/LConn2 -- _CN_88389243_400000_CN_20851038_400000/LConn2
  Nursling_Mannington_CN_23988786_400000_CN_20851038_400000/RConn3 -- T_20851038_400000;132000_Lovedean_Substation/LConn3 -- _CN_23300984_400000_CN_20851038_400000/LConn3 -- bus80/LConn1 -- Bolney_Lovedean_CN_91082448_400000_CN_20851038_400000/LConn3 -- _CN_88389243_400000_CN_20851038_400000/LConn3
  Nursling_Mannington_CN_23988786_400000_CN_5728891_400000/RConn1 -- T_5728891_400000_Fawley_Substation/LConn1 -- National_Grid_Chilling_Fawley_CN_23309078_400000_CN_5728891_400000/LConn1
  Nursling_Mannington_CN_23988786_400000_CN_5728891_400000/RConn2 -- T_5728891_400000_Fawley_Substation/LConn2 -- National_Grid_Chilling_Fawley_CN_23309078_400000_CN_5728891_400000/LConn2
  Nursling_Mannington_CN_23988786_400000_CN_5728891_400000/RConn3 -- T_5728891_400000_Fawley_Substation/LConn3 -- National_Grid_Chilling_Fawley_CN_23309078_400000_CN_5728891_400000/LConn3 -- bus81/LConn1
  Nursling_Mannington_CN_23988786_400000_CN_90099036_400000/RConn1 -- T_90099036_400000;132000_Mannington_Substation/LConn1 -- National_Grid_Chickerell_Axminster_CN_49922626_400000_CN_90099036_400000/LConn1
  Nursling_Mannington_CN_23988786_400000_CN_90099036_400000/RConn2 -- T_90099036_400000;132000_Mannington_Substation/LConn2 -- National_Grid_Chickerell_Axminster_CN_49922626_400000_CN_90099036_400000/LConn2
  Nursling_Mannington_CN_23988786_400000_CN_90099036_400000/RConn3 -- T_90099036_400000;132000_Mannington_Substation/LConn3 -- National_Grid_Chickerell_Axminster_CN_49922626_400000_CN_90099036_400000/LConn3 -- bus82/LConn1
  National_Grid_Melksham_Hinkley_Point_CN_292372019_400000_CN_103915328_400000/LConn1 -- T_292372019_400000_/LConn1 -- National_Grid_Melksham_Hinkley_Point_CN_292372019_400000_CN_119616836_400000/LConn1
  National_Grid_Melksham_Hinkley_Point_CN_292372019_400000_CN_103915328_400000/LConn2 -- T_292372019_400000_/LConn2 -- National_Grid_Melksham_Hinkley_Point_CN_292372019_400000_CN_119616836_400000/LConn2
  National_Grid_Melksham_Hinkley_Point_CN_292372019_400000_CN_103915328_400000/LConn3 -- T_292372019_400000_/LConn3 -- National_Grid_Melksham_Hinkley_Point_CN_292372019_400000_CN_119616836_400000/LConn3 -- bus83/LConn1
  National_Grid_Melksham_Hinkley_Point_CN_292372019_400000_CN_103915328_400000/RConn1 -- T_103915328_400000;275000;132000_Melksham_Substation/LConn1 -- National_Grid_Bramley_Melksham_CN_103915328_400000_CN_32796576_400000/LConn1 -- _CN_95279334_400000_CN_103915328_400000/LConn1 -- National_Grid_Melksham_?_CN_103915328_400000_CN_103962437_400000/RConn1 -- National_Grid_Melksham_?_CN_103915328_400000_CN_4911067_400000/LConn1
  National_Grid_Melksham_Hinkley_Point_CN_292372019_400000_CN_103915328_400000/RConn2 -- T_103915328_400000;275000;132000_Melksham_Substation/LConn2 -- National_Grid_Bramley_Melksham_CN_103915328_400000_CN_32796576_400000/LConn2 -- _CN_95279334_400000_CN_103915328_400000/LConn2 -- National_Grid_Melksham_?_CN_103915328_400000_CN_103962437_400000/RConn2 -- National_Grid_Melksham_?_CN_103915328_400000_CN_4911067_400000/LConn2
  National_Grid_Melksham_Hinkley_Point_CN_292372019_400000_CN_103915328_400000/RConn3 -- T_103915328_400000;275000;132000_Melksham_Substation/LConn3 -- National_Grid_Bramley_Melksham_CN_103915328_400000_CN_32796576_400000/LConn3 -- bus84/LConn1 -- _CN_95279334_400000_CN_103915328_400000/LConn3 -- National_Grid_Melksham_?_CN_103915328_400000_CN_103962437_400000/RConn3 -- National_Grid_Melksham_?_CN_103915328_400000_CN_4911067_400000/LConn3
  National_Grid_Melksham_Hinkley_Point_CN_292372019_400000_CN_119616836_400000/RConn1 -- T_119616836_400000;132000_Taunton_Substation/LConn1 -- _CN_143791249_400000_CN_119616836_400000/RConn1 -- National_Grid_Exeter_Alverdiscott_CN_26678829_400000_CN_119616836_400000/LConn1
  National_Grid_Melksham_Hinkley_Point_CN_292372019_400000_CN_119616836_400000/RConn2 -- T_119616836_400000;132000_Taunton_Substation/LConn2 -- _CN_143791249_400000_CN_119616836_400000/RConn2 -- National_Grid_Exeter_Alverdiscott_CN_26678829_400000_CN_119616836_400000/LConn2
  National_Grid_Melksham_Hinkley_Point_CN_292372019_400000_CN_119616836_400000/RConn3 -- T_119616836_400000;132000_Taunton_Substation/LConn3 -- _CN_143791249_400000_CN_119616836_400000/RConn3 -- National_Grid_Exeter_Alverdiscott_CN_26678829_400000_CN_119616836_400000/LConn3 -- bus85/LConn1
  T_304620087_400000_/LConn1 -- _CN_304620087_400000_CN_308653843_400000/RConn1
  T_304620087_400000_/LConn2 -- _CN_304620087_400000_CN_308653843_400000/RConn2
  _CN_304620087_400000_CN_308653843_400000/RConn3 -- T_304620087_400000_/LConn3 -- bus86/LConn1
  _CN_102549055_400000_CN_103150854_400000/LConn1 -- T_102549055_400000;275000_/LConn1 -- _CN_102549055_400000_CN_23228362_400000/LConn1
  _CN_102549055_400000_CN_103150854_400000/LConn2 -- T_102549055_400000;275000_/LConn2 -- _CN_102549055_400000_CN_23228362_400000/LConn2
  _CN_102549055_400000_CN_103150854_400000/LConn3 -- T_102549055_400000;275000_/LConn3 -- _CN_102549055_400000_CN_23228362_400000/LConn3 -- bus87/LConn1
  _CN_102549055_400000_CN_103150854_400000/RConn1 -- T_103150854_400000;275000_West_Thurrock_Substation/LConn1 -- West_Thurrock_?_CN_103150854_400000_CN_16582436_400000/LConn1
  _CN_102549055_400000_CN_103150854_400000/RConn2 -- T_103150854_400000;275000_West_Thurrock_Substation/LConn2 -- West_Thurrock_?_CN_103150854_400000_CN_16582436_400000/LConn2
  _CN_102549055_400000_CN_103150854_400000/RConn3 -- T_103150854_400000;275000_West_Thurrock_Substation/LConn3 -- West_Thurrock_?_CN_103150854_400000_CN_16582436_400000/LConn3 -- bus88/LConn1
  _CN_102549055_400000_CN_23228362_400000/RConn1 -- T_23228362_400000_West_Ham_Substation/LConn1 -- _CN_371757485_400000_CN_23228362_400000/LConn1
  _CN_102549055_400000_CN_23228362_400000/RConn2 -- T_23228362_400000_West_Ham_Substation/LConn2 -- _CN_371757485_400000_CN_23228362_400000/LConn2
  _CN_102549055_400000_CN_23228362_400000/RConn3 -- T_23228362_400000_West_Ham_Substation/LConn3 -- _CN_371757485_400000_CN_23228362_400000/LConn3 -- bus89/LConn1
  National_Grid_Sellindge_Dungeness_CN_23281217_400000_CN_88540693_400000/LConn1 -- T_23281217_400000_Sellindge_Converter_Station/LConn1 -- National_Grid_Canterbury_North_Sellindge_CN_23281217_400000_CN_87953830_400000/LConn1
  National_Grid_Sellindge_Dungeness_CN_23281217_400000_CN_88540693_400000/LConn2 -- T_23281217_400000_Sellindge_Converter_Station/LConn2 -- National_Grid_Canterbury_North_Sellindge_CN_23281217_400000_CN_87953830_400000/LConn2
  National_Grid_Sellindge_Dungeness_CN_23281217_400000_CN_88540693_400000/LConn3 -- T_23281217_400000_Sellindge_Converter_Station/LConn3 -- National_Grid_Canterbury_North_Sellindge_CN_23281217_400000_CN_87953830_400000/LConn3 -- bus90/LConn1
  National_Grid_Sellindge_Dungeness_CN_23281217_400000_CN_88540693_400000/RConn1 -- G_88540693_Dungeness_Nuclear_Power_Station/RConn1 -- Dungeness_Ninfield_CN_28691559_400000_CN_88540693_400000/LConn1 -- _CN_264102298_400000_CN_88540693_400000/LConn1
  National_Grid_Sellindge_Dungeness_CN_23281217_400000_CN_88540693_400000/RConn2 -- G_88540693_Dungeness_Nuclear_Power_Station/RConn2 -- Dungeness_Ninfield_CN_28691559_400000_CN_88540693_400000/LConn2 -- _CN_264102298_400000_CN_88540693_400000/LConn2
  National_Grid_Sellindge_Dungeness_CN_23281217_400000_CN_88540693_400000/RConn3 -- G_88540693_Dungeness_Nuclear_Power_Station/RConn3 -- Dungeness_Ninfield_CN_28691559_400000_CN_88540693_400000/LConn3 -- _CN_264102298_400000_CN_88540693_400000/LConn3 -- bus91/LConn1
  National_Grid_Canterbury_North_Sellindge_CN_23281217_400000_CN_87953830_400000/RConn1 -- T_87953830_400000_Canterbury_North_Substation/LConn1 -- National_Grid_Canterbury_North_Kemsley_CN_264104518_400000_CN_87953830_400000/LConn1
  National_Grid_Canterbury_North_Sellindge_CN_23281217_400000_CN_87953830_400000/RConn2 -- T_87953830_400000_Canterbury_North_Substation/LConn2 -- National_Grid_Canterbury_North_Kemsley_CN_264104518_400000_CN_87953830_400000/LConn2
  National_Grid_Canterbury_North_Sellindge_CN_23281217_400000_CN_87953830_400000/RConn3 -- T_87953830_400000_Canterbury_North_Substation/LConn3 -- National_Grid_Canterbury_North_Kemsley_CN_264104518_400000_CN_87953830_400000/LConn3 -- bus92/LConn1
  National_Grid_Chickerell_Axminster_CN_49922626_400000_CN_26678829_400000/LConn1 -- T_49922626_400000;132000_Chickerell_Substation/LConn1 -- National_Grid_Chickerell_Axminster_CN_49922626_400000_CN_90099036_400000/RConn1 -- National_Grid_Chickerell_Axminster_CN_49922626_400000_CN_34205588_400000/LConn1
  National_Grid_Chickerell_Axminster_CN_49922626_400000_CN_26678829_400000/LConn2 -- T_49922626_400000;132000_Chickerell_Substation/LConn2 -- National_Grid_Chickerell_Axminster_CN_49922626_400000_CN_90099036_400000/RConn2 -- National_Grid_Chickerell_Axminster_CN_49922626_400000_CN_34205588_400000/LConn2
  National_Grid_Chickerell_Axminster_CN_49922626_400000_CN_26678829_400000/LConn3 -- T_49922626_400000;132000_Chickerell_Substation/LConn3 -- National_Grid_Chickerell_Axminster_CN_49922626_400000_CN_90099036_400000/RConn3 -- bus93/LConn1 -- National_Grid_Chickerell_Axminster_CN_49922626_400000_CN_34205588_400000/LConn3
  National_Grid_Chickerell_Axminster_CN_49922626_400000_CN_26678829_400000/RConn1 -- T_26678829_400000;132000_Exeter_Substation/LConn1 -- _CN_26678829_400000_CN_26938722_400000/LConn1 -- National_Grid_Exeter_Alverdiscott_CN_26678829_400000_CN_119616836_400000/RConn1
  National_Grid_Chickerell_Axminster_CN_49922626_400000_CN_26678829_400000/RConn2 -- T_26678829_400000;132000_Exeter_Substation/LConn2 -- _CN_26678829_400000_CN_26938722_400000/LConn2 -- National_Grid_Exeter_Alverdiscott_CN_26678829_400000_CN_119616836_400000/RConn2
  National_Grid_Chickerell_Axminster_CN_49922626_400000_CN_26678829_400000/RConn3 -- T_26678829_400000;132000_Exeter_Substation/LConn3 -- _CN_26678829_400000_CN_26938722_400000/LConn3 -- National_Grid_Exeter_Alverdiscott_CN_26678829_400000_CN_119616836_400000/RConn3 -- bus94/LConn1
  T_34205588_400000;132000_Axminster_Substation/LConn1 -- National_Grid_Chickerell_Axminster_CN_49922626_400000_CN_34205588_400000/RConn1
  T_34205588_400000;132000_Axminster_Substation/LConn2 -- National_Grid_Chickerell_Axminster_CN_49922626_400000_CN_34205588_400000/RConn2
  National_Grid_Chickerell_Axminster_CN_49922626_400000_CN_34205588_400000/RConn3 -- T_34205588_400000;132000_Axminster_Substation/LConn3 -- bus95/LConn1
  National_Grid_Canterbury_North_Kemsley_CN_264104518_400000_CN_91010022_400000/LConn1 -- T_264104518_400000;132000_Cleve_Hill_Substation/LConn1 -- National_Grid_Canterbury_North_Kemsley_CN_264104518_400000_CN_87953830_400000/RConn1
  National_Grid_Canterbury_North_Kemsley_CN_264104518_400000_CN_91010022_400000/LConn2 -- T_264104518_400000;132000_Cleve_Hill_Substation/LConn2 -- National_Grid_Canterbury_North_Kemsley_CN_264104518_400000_CN_87953830_400000/RConn2
  National_Grid_Canterbury_North_Kemsley_CN_264104518_400000_CN_91010022_400000/LConn3 -- T_264104518_400000;132000_Cleve_Hill_Substation/LConn3 -- National_Grid_Canterbury_North_Kemsley_CN_264104518_400000_CN_87953830_400000/RConn3 -- bus96/LConn1
  National_Grid_Canterbury_North_Kemsley_CN_264104518_400000_CN_91010022_400000/RConn1 -- T_91010022_400000;132000_Kemsley_Substation/LConn1 -- National_Grid_Northfleet_West_Rowdown_CN_23299657_400000_CN_91010022_400000/LConn1 -- National_Grid_Grain_Kemsley_CN_109189893_400000_CN_91010022_400000/RConn1
  National_Grid_Canterbury_North_Kemsley_CN_264104518_400000_CN_91010022_400000/RConn2 -- T_91010022_400000;132000_Kemsley_Substation/LConn2 -- National_Grid_Northfleet_West_Rowdown_CN_23299657_400000_CN_91010022_400000/LConn2 -- National_Grid_Grain_Kemsley_CN_109189893_400000_CN_91010022_400000/RConn2
  National_Grid_Canterbury_North_Kemsley_CN_264104518_400000_CN_91010022_400000/RConn3 -- T_91010022_400000;132000_Kemsley_Substation/LConn3 -- National_Grid_Northfleet_West_Rowdown_CN_23299657_400000_CN_91010022_400000/LConn3 -- National_Grid_Grain_Kemsley_CN_109189893_400000_CN_91010022_400000/RConn3 -- bus97/LConn1
  T_23299657_400000_Rowdown_Substation/LConn1 -- National_Grid_Northfleet_West_Rowdown_CN_23299657_400000_CN_91010022_400000/RConn1
  T_23299657_400000_Rowdown_Substation/LConn2 -- National_Grid_Northfleet_West_Rowdown_CN_23299657_400000_CN_91010022_400000/RConn2
  National_Grid_Northfleet_West_Rowdown_CN_23299657_400000_CN_91010022_400000/RConn3 -- T_23299657_400000_Rowdown_Substation/LConn3 -- bus98/LConn1
  _CN_93878866_400000_CN_293585871_400000/LConn1 -- T_93878866__/LConn1 -- _CN_93878866_400000_CN_93878867_400000/LConn1
  _CN_93878866_400000_CN_293585871_400000/LConn2 -- T_93878866__/LConn2 -- _CN_93878866_400000_CN_93878867_400000/LConn2
  _CN_93878866_400000_CN_293585871_400000/LConn3 -- T_93878866__/LConn3 -- _CN_93878866_400000_CN_93878867_400000/LConn3 -- bus99/LConn1
  _CN_93878866_400000_CN_293585871_400000/RConn1 -- T_293585871__/LConn1 -- _CN_293585871_400000_CN_293585872_400000/LConn1
  _CN_93878866_400000_CN_293585871_400000/RConn2 -- T_293585871__/LConn2 -- _CN_293585871_400000_CN_293585872_400000/LConn2
  _CN_93878866_400000_CN_293585871_400000/RConn3 -- T_293585871__/LConn3 -- _CN_293585871_400000_CN_293585872_400000/LConn3 -- bus100/LConn1
  _CN_93878866_400000_CN_93878867_400000/RConn1 -- T_93878867_400000;132000_/LConn1 -- National_Grid_Macclesfield_?_CN_92419253_400000_CN_93878867_400000/LConn1
  _CN_93878866_400000_CN_93878867_400000/RConn2 -- T_93878867_400000;132000_/LConn2 -- National_Grid_Macclesfield_?_CN_92419253_400000_CN_93878867_400000/LConn2
  _CN_93878866_400000_CN_93878867_400000/RConn3 -- T_93878867_400000;132000_/LConn3 -- National_Grid_Macclesfield_?_CN_92419253_400000_CN_93878867_400000/LConn3 -- bus101/LConn1
  _CN_41809491_400000_CN_89453364_400000/LConn1 -- T_41809491_400000_Sundon_Substation/LConn1 -- _CN_41809491_400000_CN_24165071_400000/RConn1 -- _CN_41809491_400000_CN_4746208_400000/LConn1
  _CN_41809491_400000_CN_89453364_400000/LConn2 -- T_41809491_400000_Sundon_Substation/LConn2 -- _CN_41809491_400000_CN_24165071_400000/RConn2 -- _CN_41809491_400000_CN_4746208_400000/LConn2
  _CN_41809491_400000_CN_89453364_400000/LConn3 -- T_41809491_400000_Sundon_Substation/LConn3 -- _CN_41809491_400000_CN_24165071_400000/RConn3 -- bus102/LConn1 -- _CN_41809491_400000_CN_4746208_400000/LConn3
  _CN_41809491_400000_CN_89453364_400000/RConn1 -- T_89453364_400000_/LConn1 -- _CN_23059230_400000_CN_89453364_400000/RConn1
  _CN_41809491_400000_CN_89453364_400000/RConn2 -- T_89453364_400000_/LConn2 -- _CN_23059230_400000_CN_89453364_400000/RConn2
  _CN_41809491_400000_CN_89453364_400000/RConn3 -- T_89453364_400000_/LConn3 -- _CN_23059230_400000_CN_89453364_400000/RConn3 -- bus103/LConn1
  T_4746208_400000;275000;132000_Elstree_Substation/LConn1 -- _CN_41809491_400000_CN_4746208_400000/RConn1
  T_4746208_400000;275000;132000_Elstree_Substation/LConn2 -- _CN_41809491_400000_CN_4746208_400000/RConn2
  _CN_41809491_400000_CN_4746208_400000/RConn3 -- T_4746208_400000;275000;132000_Elstree_Substation/LConn3 -- bus104/LConn1
  T_142841192_400000;275000;132000_Bradford_West_Substation/LConn1 -- _CN_55578199_400000_CN_142841192_400000/RConn1
  T_142841192_400000;275000;132000_Bradford_West_Substation/LConn2 -- _CN_55578199_400000_CN_142841192_400000/RConn2
  _CN_55578199_400000_CN_142841192_400000/RConn3 -- T_142841192_400000;275000;132000_Bradford_West_Substation/LConn3 -- bus105/LConn1
  _CN_55578199_400000_CN_90547674_400000/RConn1 -- T_90547674_400000;275000_Monk_Fryston_substation/LConn1 -- _CN_313495269_400000_CN_90547674_400000/LConn1
  _CN_55578199_400000_CN_90547674_400000/RConn2 -- T_90547674_400000;275000_Monk_Fryston_substation/LConn2 -- _CN_313495269_400000_CN_90547674_400000/LConn2
  _CN_55578199_400000_CN_90547674_400000/RConn3 -- T_90547674_400000;275000_Monk_Fryston_substation/LConn3 -- _CN_313495269_400000_CN_90547674_400000/LConn3 -- bus106/LConn1
  _CN_143219044_400000_CN_284874050_400000/RConn1 -- T_143219044_400000;132000_Gretna_Substation/LConn1 -- _CN_143219044_400000_CN_88799419_400000/LConn1
  _CN_143219044_400000_CN_284874050_400000/RConn2 -- T_143219044_400000;132000_Gretna_Substation/LConn2 -- _CN_143219044_400000_CN_88799419_400000/LConn2
  _CN_143219044_400000_CN_284874050_400000/RConn3 -- T_143219044_400000;132000_Gretna_Substation/LConn3 -- _CN_143219044_400000_CN_88799419_400000/LConn3 -- bus107/LConn1
  _CN_143219044_400000_CN_88799419_400000/RConn1 -- T_88799419_400000;275000;132000_Harker_Substation/LConn1 -- _CN_45357172_400000_CN_88799419_400000/LConn1
  _CN_143219044_400000_CN_88799419_400000/RConn2 -- T_88799419_400000;275000;132000_Harker_Substation/LConn2 -- _CN_45357172_400000_CN_88799419_400000/LConn2
  _CN_143219044_400000_CN_88799419_400000/RConn3 -- T_88799419_400000;275000;132000_Harker_Substation/LConn3 -- _CN_45357172_400000_CN_88799419_400000/LConn3 -- bus108/LConn1
